simulink model "pd_plus_testings_7DOF_alternative"  (R2022b)
settings: Solver=ode4  StartTime=0.0  StopTime=101  FixedStep=1e-3  RelTol=1e-3
InitFcn:
  | parameters_7dof;
undefined symbols (not defined in the file): param_robot, q_0
(part 6 of 7)

== matlab function pd_plus_testings_7DOF_alternative/Subsystem/Coriolis Matrix ==
  data: q_state input; C output; q_state_dot input
function C = Franka_CoriolisMatrix(q_state, q_state_dot)
% Author: TU Wien, ACIN Robotics group
% Optimized and generated from Maple

  C = zeros(7,7);
  t2638 = q_state(7);
  t2624 = cos(t2638);
  t3209 = 0.10967182128164640000000000000000e-2 * t2624;
  t2617 = sin(t2638);
  t3260 = 0.33449653235675560000000000000000e-2 * t2617;
  t2102 = t3209 + t3260;
  t1973 = t2102 + 0.18713819462921000000000000000000e-3;
  t2639 = q_state(6);
  t2618 = sin(t2639);
  t3973 = t1973 * t2618;
  t1810 = t3973 - 0.30304889466540600000000000000000e-2;
  t3252 = 0.11357396418885000000000000000000e-1 * t2618;
  t2171 = -0.24178658687700000000000000000000e-2 + t3252;
  t2640 = q_state(5);
  t2619 = sin(t2640);
  t3206 = 0.12763550042100000000000000000000e-2 * t2624;
  t3271 = 0.51602752476000000000000000000000e-3 * t2617;
  t3723 = -t3271 - t3206;
  t3047 = -0.27219646194675000000000000000000e-1 + t3723;
  t2156 = 0.48418875570424600000000000000000e-2 * t2617 + 0.55042935974400000000000000000000e-3;
  t2610 = t2624 ^ 2;
  t2388 = 0.15804348732630080000000000000000e-2 * t2610;
  t2412 = 0.13614453378240000000000000000000e-2 * t2617;
  t3020 = 0.5826996021941340000000000000000e-3 - t2388 - t2412;
  t1748 = t2156 * t2624 + t3020;
  t4010 = t1748 * t2619;
  t1556 = t3047 - t4010;
  t2625 = cos(t2639);
  t4368 = t1556 * t2625;
  t1365 = t1810 * t2619 - t2171 + t4368;
  t2641 = q_state(4);
  t2627 = cos(t2641);
  t2613 = t2627 ^ 2;
  t4376 = t1365 * t2613;
  t2626 = cos(t2640);
  t4375 = t1365 * t2626;
  t2024 = t2102 + 0.187138194629210e-3;
  t1841 = t2024 * t2619 - 0.11357396418885000000000000000000e-1;
  t1801 = t1841 * t2625;
  t3249 = 0.52863517876992000000000000000000e-1 * t2618;
  t4130 = -0.33449653235675560000000000000000e-2 * t2624 + 0.10967182128164640000000000000000e-2 * t2617;
  t1838 = -t4130 + t3249 + 0.8968493211292842000000000000000e-2;
  t2107 = -0.66899306471351120000000000000000e-2 * t2624 + 0.21934364256329280000000000000000e-2 * t2617;
  t1967 = 0.22044137530701260000000000000000e-1 - t2107;
  t2611 = t2625 ^ 2;
  t3977 = t1967 * t2611;
  t3510 = t1838 - t3977;
  t2382 = 0.48152918111602840000000000000000e-2 * t2610;
  t3265 = 0.15804348732630080000000000000000e-2 * t2617;
  t2160 = -0.27228906756480000000000000000000e-2 + t3265;
  t2416 = 0.11008587194880000000000000000000e-2 * t2617;
  t2603 = t2617 ^ 2;
  t3573 = -t2160 * t2624 + t2416 + 0.26595745882176000000000000000000e-4 * t2603;
  t2986 = -0.11560955249855324000000000000000e-1 - t3573;
  t1663 = t2382 + t2986;
  t3194 = 0.59408523832320000000000000000000e-2 * t2624;
  t3262 = 0.24018735697920000000000000000000e-2 * t2617;
  t3718 = -t3262 - t3194;
  t3046 = -0.12669508046976000000000000000000e0 + t3718;
  t1513 = t1663 * t2618 + t3046;
  t4044 = t1513 * t2625;
  t1348 = t3510 - t4044;
  t4374 = t1348 * t2626;
  t4169 = -t4374 + t1801;
  t3201 = 0.24018735697920000000000000000000e-2 * t2624;
  t3729 = 0.59408523832320000000000000000000e-2 * t2617 - t3201;
  t4300 = 0.47796540830203740000000000000000e-1 - t3729;
  t4369 = t1556 * t2618;
  t2890 = t2619 * t4300 + t4169 - t4369 + 0.27752814537092170000000000000000e0;
  t4047 = t1348 * t2619;
  t3717 = -0.66899306471351120000000000000000e-2 * t2617 - 0.21934364256329280000000000000000e-2 * t2624;
  t2036 = t3717 * t2611;
  t2822 = t2036 + t2102;
  t3208 = 0.11008587194880000000000000000000e-2 * t2624;
  t3257 = 0.96837751140849200000000000000000e-2 * t2617;
  t2247 = t2624 * t3257;
  t3739 = -t2247 + t2388;
  t1704 = t2160 * t2617 + t3208 - t3739;
  t4326 = t1704 * t2618 - t3729;
  t4035 = t2625 * t4326;
  t4359 = t2822 - t4035;
  t1392 = t4359 * t2626;
  t2381 = 0.48418875570424600000000000000000e-2 * t2610;
  t3261 = 0.31608697465260160000000000000000e-2 * t2617;
  t2248 = t2624 * t3261;
  t2473 = 0.13614453378240000000000000000000e-2 * t2624;
  t3749 = t2248 - t2473;
  t1706 = -t2156 * t2617 + t2381 + t3749;
  t2413 = 0.12763550042100000000000000000000e-2 * t2617;
  t2480 = 0.51602752476000000000000000000000e-3 * t2624;
  t2111 = t2413 - t2480;
  t1564 = t1706 * t2619 - t2111;
  t4373 = -t1564 * t2618 - t1392;
  t2620 = sin(t2641);
  t1418 = t1513 * t2620 - t3047;
  t4046 = t1418 * t2625;
  t4372 = -t2171 - t4046;
  t2643 = q_state(2);
  t2629 = cos(t2643);
  t2642 = q_state(3);
  t2621 = sin(t2642);
  t2628 = cos(t2642);
  t2524 = 0.60149e-1 * t2625 + 0.14117e-1 * t2618;
  t3551 = 0.10517e-1 * t2626;
  t3300 = t2524 * t2619 + t3551;
  t2521 = 0.60149e-1 * t2618 - 0.14117e-1 * t2625;
  t2354 = t2521 + 0.384e0;
  t2226 = t2354 * t2620;
  t3558 = 0.10517e-1 * t2619;
  t2875 = -t2524 * t2626 + t3558;
  t2828 = 0.825e-1 + t2875;
  t4312 = t2627 * t2828;
  t3354 = -t2226 - t4312;
  t4331 = -0.825e-1 - t3354;
  t4341 = t2621 * t3300 + t2628 * t4331;
  t4250 = t2629 * t4341;
  t2622 = sin(t2643);
  t4237 = t4341 * t2622;
  t4001 = t1841 * t2618;
  t4370 = -t4001 - t4368;
  t4347 = t1748 * t2618;
  t1557 = t4300 + t4347;
  t1538 = t1557 * t2619;
  t2401 = 0.4815291811160284000000000000000e-2 * t2610;
  t2982 = 0.17806630741175110000000000000000e-1 + t3573;
  t1682 = t2982 - t2401;
  t3832 = t2618 * t2625;
  t4367 = (0.2e1 * t1682 - 0.12491350982639572000000000000000e-1) * t3832;
  t1664 = t2382 - t2982;
  t4366 = (0.2e1 * t1664 + 0.12491350982639572000000000000000e-1) * t3832;
  t3835 = t2618 * t2619;
  t4365 = (t1564 * t2625 + t3835 * t4130) * t2626;
  t2235 = 0.187138194629210e-3 + t3260;
  t3513 = t2625 * t3209 + t4347;
  t4364 = t2235 * t2625 + t3513;
  t2157 = 0.18713819462921000000000000000000e-3 + t3260;
  t4363 = t2157 * t2625 + t3513;
  t3694 = t1967 * t3832;
  t4025 = t1682 * t2611;
  t3319 = -t3694 - t4025;
  t2159 = 0.24209437785212300000000000000000e-2 * t2617 + 0.27521467987200000000000000000000e-3;
  t3898 = t2159 * t2617;
  t3204 = 0.15804348732630080000000000000000e-2 * t2624;
  t2249 = t2617 * t3204;
  t2385 = 0.24209437785212300000000000000000e-2 * t2610;
  t2477 = 0.68072266891200000000000000000000e-3 * t2624;
  t2854 = t2477 - t2385;
  t4210 = t2249 - t2854;
  t1707 = -t3898 + t4210;
  t4196 = t1707 * t2625;
  t4241 = t4130 * t2618;
  t1524 = t1706 * t2625 + t4241;
  t2612 = t2626 ^ 2;
  t4334 = t1524 * t2612;
  t4362 = t4334 - t4196;
  t3532 = 0.345563e0 * t2627;
  t3120 = 0.41065e-1 * t2619 + 0.11953e-1 * t2626;
  t2356 = t3120 + 0.825e-1;
  t3871 = t2356 * t2620;
  t3295 = -t3532 + t3871;
  t2046 = t3295 - 0.316e0;
  t2571 = 0.345563e0 * t2620;
  t3870 = t2356 * t2627;
  t4135 = t2571 + t3870;
  t4207 = -0.825e-1 + t4135;
  t2004 = t4207 * t2628;
  t3549 = 0.41065e-1 * t2626;
  t2522 = 0.11953e-1 * t2619 - t3549;
  t3820 = t2621 * t2522;
  t1785 = t2004 - t3820;
  t4002 = t1785 * t2622;
  t1578 = t2046 * t2629 - t4002;
  t2644 = q_state(1);
  t2630 = cos(t2644);
  t3160 = 0.61297300000000000000000000000000e0 * t2630;
  t3102 = t1578 * t3160;
  t4361 = 0.1e1 * t3102;
  t4358 = -t1524 * t2626 + t3723;
  t2604 = t2618 ^ 2;
  t2374 = 0.62456754913197860000000000000000e-2 * t2604;
  t3578 = t2249 + 0.16270818883971600000000000000000e-3 * t2603 - t2374;
  t1360 = t1664 * t2611 + t3578 + 0.50045957458821760000000000000000e-2 * t2610 - 0.12569364734109380000000000000000e-2 - t3694;
  t2033 = t2111 * t2618;
  t4342 = t1706 * t2618 + t3718;
  t4356 = -t2619 * t4342 + t2033;
  t2098 = 0.10517000000000000000000000000000e-1 * t2617 - 0.42520000000000000000000000000000e-2 * t2624;
  t2037 = t2098 * t2619;
  t2128 = 0.10517000000000000000000000000000e-1 * t2624 + 0.42520000000000000000000000000000e-2 * t2617;
  t1966 = 0.88000000000000000000000000000000e-1 + t2128;
  t3248 = 0.61597000000000000000000000000000e-1 * t2618;
  t3793 = t2625 * t2626;
  t3760 = t1966 * t3793 + t2626 * t3248;
  t4156 = t2037 + t3760;
  t1561 = 0.82500000000000000000000000000000e-1 - t4156;
  t4353 = t1561 * t2620;
  t4352 = t1561 * t2627;
  t3972 = t1973 * t2625;
  t4350 = t3972 + t4347;
  t4346 = t1748 * t2625;
  t1506 = t4346 - t1810;
  t2523 = 0.39252e-1 * t2628 + 0.27518e-1 * t2621;
  t2623 = sin(t2644);
  t3117 = 0.39252e-1 * t2621 - 0.27518e-1 * t2628;
  t2871 = t3117 * t2629 - 0.249498e0 * t2622;
  t4324 = t2523 * t2623 + t2630 * t2871;
  t4349 = 0.1e1 * t4324;
  t4322 = 0.1e1 * t2623;
  t3897 = t2159 * t2624;
  t2390 = 0.79021743663150400000000000000000e-3 * t2610;
  t2419 = 0.68072266891200000000000000000000e-3 * t2617;
  t2883 = -0.29134980109706700000000000000000e-3 + t2419;
  t4133 = t2883 + t2390;
  t1744 = t3897 - t4133;
  t2423 = 0.25801376238000000000000000000000e-3 * t2617;
  t2478 = 0.63817750210500000000000000000000e-3 * t2624;
  t3724 = t2423 + t2478;
  t1962 = -t3724 - 0.13609823097337500000000000000000e-1;
  t3985 = t1962 * t2619;
  t1549 = t1744 - t3985;
  t4348 = t1549 * t2625;
  t1643 = t1663 * t2611;
  t3958 = t3047 * t2625;
  t1755 = t3958 - t2171;
  t4345 = t1755 * t2619;
  t1726 = t1755 * t2626;
  t4344 = t1785 * t2629;
  t3791 = t2626 * t2620;
  t2420 = 0.63817750210500000000000000000000e-3 * t2617;
  t3216 = 0.25801376238000000000000000000000e-3 * t2624;
  t2119 = t3216 - t2420;
  t3044 = -0.55993270925625000000000000000000e-2 - t2119;
  t4343 = t3044 * t2626;
  t1552 = -t2619 * t3047 + t1748;
  t1672 = t1704 * t2611;
  t2001 = t3717 * t3832;
  t3317 = -t2001 - t1672;
  t3789 = t2626 * t2628;
  t4340 = 0.1e1 * t3789;
  t4339 = 0.1e1 * t4345;
  t3263 = 0.23920000000000000000000000000000e-2 * t2617;
  t2338 = 0.682e-3 + t3263;
  t3205 = 0.14820000000000000000000000000000e-2 * t2624;
  t2387 = 0.17120000000000000000000000000000e-2 * t2610;
  t3838 = t2617 * t2624;
  t3087 = 0.49780000000000000000000000000000e-2 * t3838;
  t2826 = t3087 - t2387;
  t1885 = t2826 - 0.14600000000000000000000000000000e-2;
  t3990 = t1885 * t2625;
  t3764 = -t2618 * t3205 + t3990;
  t3585 = -t2338 * t2618 + t3764;
  t1618 = 0.4234e-2 + t3585;
  t3826 = t2619 * t2626;
  t1581 = t1618 * t3826;
  t3565 = 0.5317e-1 * t2620;
  t2563 = -0.316e0 + t3565;
  t3533 = 0.104419e0 * t2627;
  t3119 = 0.104419e0 * t2620 + 0.5317e-1 * t2627;
  t2357 = t3119 - 0.825e-1;
  t2088 = t2357 * t2628 - 0.27454e-1 * t2621;
  t4259 = t2088 * t2629;
  t1767 = t4259 + t2622 * (t2563 - t3533);
  t4338 = t1767 * t2630;
  t2414 = 0.12009367848960000000000000000000e-2 * t2617;
  t2161 = t2414 + 0.63347540234880000000000000000000e-1;
  t2469 = 0.29704261916160000000000000000000e-2 * t2624;
  t1978 = -t2469 - t2161;
  t4337 = t1978 * t2625;
  t3091 = 0.17120000000000000000000000000000e-2 * t3838;
  t3273 = 0.49780000000000000000000000000000e-2 * t2610;
  t2825 = t3091 + t3273;
  t1897 = 0.5644000000000000000000000000000e-2 + t2825;
  t1854 = t1897 * t2611;
  t2848 = -0.47840000000000000000000000000000e-2 * t2624 + 0.29640000000000000000000000000000e-2 * t2617;
  t2065 = -0.436e-3 + t2848;
  t1948 = t2065 * t3832;
  t3762 = t1854 + t1948;
  t1486 = t2825 + t3762 - 0.5410000000000000000000000000000e-2;
  t2605 = t2619 ^ 2;
  t3711 = -0.1e1 * t2605 + t2612;
  t4336 = t3711 * t1486;
  t2422 = 0.54835910640823200000000000000000e-3 * t2617;
  t3203 = 0.16724826617837780000000000000000e-2 * t2624;
  t2852 = -t3203 + t2422;
  t4248 = t2852 * t2618;
  t4335 = t4248 * t2627;
  t3289 = 0.4841887557042460000000000000000e-2 * t2617;
  t2200 = 0.55042935974400000000000000000000e-3 + t3289;
  t1749 = -t2200 * t2624 - t3020;
  t1559 = -t1749 * t2618 + t4300;
  t4333 = t1559 + t3972;
  t4319 = t1707 * t2619;
  t4332 = t2119 + t4319;
  t3269 = 0.79021743663150400000000000000000e-3 * t2617;
  t2250 = t2624 * t3269;
  t3748 = t2250 + 0.25022978729410880000000000000000e-2 * t2610;
  t3121 = 0.6284682367054690000000000000000e-3 - t3748;
  t4330 = 0.81354094419858000000000000000000e-4 * t2603 - t3121;
  t2002 = 0.3742763892584200000000000000000e-3 - t3717;
  t3953 = t2002 * t2625;
  t2155 = 0.11008587194880000000000000000000e-2 + t3257;
  t2383 = 0.31608697465260160000000000000000e-2 * t2610;
  t2408 = 0.27228906756480000000000000000000e-2 * t2617;
  t4282 = t2383 + t2408 - 0.11653992043882680000000000000000e-2;
  t1742 = -t2155 * t2624 + t4282;
  t4318 = t1742 * t2618;
  t4329 = t3953 - t4318;
  t3932 = t2620 * t2828;
  t4328 = t3932 - 0.316e0;
  t3552 = 0.61597e-1 * t2625;
  t2527 = 0.10517e-1 * t2624 + 0.4252e-2 * t2617;
  t2359 = t2527 + 0.88e-1;
  t3869 = t2359 * t2618;
  t2834 = -t3552 + t3869;
  t4105 = 0.384e0 + t2834;
  t4242 = t4105 * t2627;
  t4274 = -t4242 - 0.316e0;
  t4243 = t4105 * t2620;
  t4106 = 0.825e-1 - t4243;
  t4327 = t1486 * t3826 + t3585 + 0.6898e-2;
  t1968 = 0.11022068765350630000000000000000e-1 - t4130;
  t2421 = 0.55042935974400000000000000000000e-3 * t2617;
  t3725 = t2421 + t2473;
  t1971 = 0.89166132435286430000000000000000e-2 + t3725;
  t3790 = t2626 * t2627;
  t1603 = t1968 * t3790 - t1971 * t2620;
  t2168 = 0.76800000000000000000000000000000e0 * t2618 + 0.17600000000000000000000000000000e0;
  t2410 = 0.24444132201840000000000000000000e-2 * t2617;
  t3211 = 0.98827089590400000000000000000000e-3 * t2624;
  t4222 = -t3211 + t2410;
  t2812 = t2618 * t4222;
  t3451 = 0.7735484874e-2 * t2617;
  t3834 = t2618 * t2620;
  t4323 = t2119 * t3834 + t2168 * t3451 + t2627 * t2812;
  t2306 = t2625 * t3205;
  t3991 = t1885 * t2618;
  t1623 = t2338 * t2625 + t2306 + t3991;
  t4321 = t1623 * t3826;
  t4320 = t1707 * t2618;
  t4317 = t1744 * t2618;
  t1720 = t1744 * t2619;
  t4316 = t1744 * t2620;
  t4315 = t1744 * t2621;
  t4016 = t1744 * t2625;
  t4014 = t1744 * t2626;
  t3786 = t2627 * t2625;
  t4314 = t1744 * t3786;
  t3787 = t2627 * t2618;
  t4313 = t1744 * t3787;
  t3548 = 0.61597e-1 * t2626;
  t2537 = t2618 * t3548;
  t3123 = 0.10517e-1 * t2617 - 0.4252e-2 * t2624;
  t4256 = t2619 * t3123;
  t4122 = -t2359 * t3793 - t4256;
  t1775 = t2537 - 0.825e-1 - t4122;
  t4005 = t1775 * t2620;
  t4004 = t1775 * t2627;
  t2509 = 0.11357396418885000000000000000000e-1 * t2625;
  t3961 = t3047 * t2618;
  t4217 = -t3961 - t2509;
  t1771 = t2626 * t4217;
  t3559 = 0.61597e-1 * t2618;
  t3301 = t2359 * t2625 + t3559;
  t4245 = t3123 * t2626;
  t2741 = t2619 * t3301 - t4245;
  t4311 = t2741 * t2621;
  t4310 = t2741 * t2628;
  t3669 = t1897 * t3832;
  t3934 = t2065 * t2611;
  t4108 = t2065 * t2604 + 0.2e1 * t3669 - t3934;
  t4309 = -t3826 * t4108 - t1623;
  t1939 = t2159 * t2618 + 0.12009367848960000000000000000000e-2;
  t2407 = 0.29704261916160000000000000000000e-2 * t2617;
  t2158 = t2407 - 0.23898270415101870000000000000000e-1;
  t2268 = t2618 * t2390;
  t1531 = t1939 * t2624 - t2618 * t2883 - t2158 - t2268;
  t2609 = t2623 ^ 2;
  t2616 = t2630 ^ 2;
  t4134 = t2616 + t2609;
  t1935 = t2002 * t2618;
  t3155 = -t1742 * t2625 + 0.60609778933081200000000000000000e-2;
  t1507 = t3155 - t1935;
  t3290 = 0.4841887557042460000000000000000e-2 * t2610;
  t4307 = -t3290 - t3749;
  t2375 = 0.31228377456598930000000000000000e-2 * t2604;
  t3747 = t2250 + t2385;
  t4306 = t3747 - t2375;
  t3053 = 0.33106000000000000000000000000000e-1 - t2825;
  t2471 = 0.23920000000000000000000000000000e-2 * t2624;
  t3266 = 0.14820000000000000000000000000000e-2 * t2617;
  t3720 = -t3266 + t2471;
  t2063 = -0.218e-3 - t3720;
  t3666 = t2063 * t3832;
  t3092 = 0.85600000000000000000000000000000e-3 * t3838;
  t3274 = 0.24890000000000000000000000000000e-2 * t2610;
  t2018 = t3092 + t3274;
  t1884 = t2018 + 0.28220000000000000000000000000000e-2;
  t3992 = t1884 * t2611;
  t3763 = -t3992 - t3666;
  t4305 = t3763 - t3053;
  t3909 = t2119 * t2627;
  t4304 = -t3909 + t2119;
  t3291 = 0.2420943778521230000000000000000e-2 * t2610;
  t3449 = 0.7735484874e-2 * t2624;
  t3347 = t2168 * t3449;
  t4302 = (t3291 + 0.790217436631504e-3 * t3838 - 0.6002993810686607000000000000000e-2) * t2612 - 0.1e1 * t3347;
  t2573 = 0.249498e0 * t2629;
  t4183 = t2622 * t3117;
  t4281 = t2573 + t4183;
  t4301 = 0.3228604e1 * t4281;
  t3214 = 0.54835910640823200000000000000000e-3 * t2624;
  t3264 = 0.16724826617837780000000000000000e-2 * t2617;
  t3719 = -t3264 - t3214;
  t2025 = -t3719 + 0.93569097314605e-4;
  t4299 = 0.1e1 * t1744;
  t4298 = t2627 - 0.1e1;
  t1813 = -t1973 * t2619 + 0.11357396418885000000000000000000e-1;
  t4296 = t1813 * t2618;
  t3275 = 0.85600000000000000000000000000000e-3 * t2610;
  t1857 = 0.85600000000000000000000000000000e-3 * t2603 + t3087 - t3275;
  t2106 = t3205 + t3263;
  t3664 = t2106 * t3832;
  t3999 = t1857 * t2611;
  t3765 = t3999 - t3664;
  t4160 = t1857 + t3765;
  t4295 = t2612 * t4160;
  t3817 = t2621 * t2620;
  t3813 = t2621 * t2627;
  t4294 = t2621 * t4207;
  t2845 = t2622 * t2875;
  t3783 = t2628 * t2627;
  t2204 = t2522 * t3783;
  t4104 = t2621 * t3120 + t2204;
  t4293 = t2622 * t4104;
  t3798 = t2625 * t2619;
  t3329 = -t2359 * t3798 - t2619 * t3559 + t4245;
  t4290 = t3329 * t2621;
  t4003 = t3329 * t2628;
  t4288 = (t2621 * t3123 + t3301 * t3783) * t2619;
  t2386 = 0.24076459055801420000000000000000e-2 * t2610;
  t3731 = -t2386 + t2421;
  t2162 = -0.13614453378240000000000000000000e-2 + t3269;
  t3892 = t2162 * t2624;
  t2980 = 0.89033153705875550000000000000000e-2 - t3892 + t3731;
  t3402 = 0.13297872941088e-4 * t2603;
  t1696 = t2980 + t3402;
  t4287 = t1696 * t2611 + 0.3122837745659893e-2 * t2604;
  t3945 = t2046 * t2622;
  t1572 = t3945 + t4344;
  t3195 = 0.48418875570424600000000000000000e-2 * t2624;
  t2827 = t2617 * t3195 - t2390;
  t3279 = 0.79021743663150400000000000000000e-3 * t2603;
  t1858 = t2827 + t3279;
  t2479 = 0.55042935974400000000000000000000e-3 * t2624;
  t3893 = t2162 * t2617;
  t1710 = -t2827 - t2479 - t3893;
  t1678 = t1710 * t2611;
  t3665 = t2102 * t3832;
  t4124 = t3665 + t1678;
  t4286 = -t1858 + t4124;
  t2027 = t2102 * t2611;
  t1677 = t1710 * t2618;
  t2474 = 0.12009367848960000000000000000000e-2 * t2624;
  t2103 = t2407 - t2474;
  t4164 = t1677 + t2103;
  t4036 = t4164 * t2625;
  t4285 = -t2027 + t4036;
  t2112 = t2414 + t2469;
  t4247 = t2852 * t2625;
  t4284 = -t2112 - t4247;
  t1940 = t2162 * t2618 - 0.29704261916160000000000000000000e-2;
  t4283 = -t1940 * t2624 + t2161;
  t1807 = 0.175156065026714e-3 - t4306;
  t3709 = -0.2e1 * t3826;
  t2179 = 0.11198654185125000000000000000000e-1 - t2413;
  t1989 = t2480 + t2179;
  t3956 = t1989 * t2626;
  t3758 = 0.46660838454822060000000000000000e-2 * t3826 + t3956;
  t4279 = t3758 + t1807 * t3709 - 0.1e1 * t4345;
  t3873 = t2354 * t2627;
  t4278 = t3873 - t3932;
  t3369 = -t3565 + t3533;
  t2355 = -t3369 - 0.316e0;
  t1791 = -t2355 * t2622 - t4259;
  t4276 = -0.1e1 * t2603 + t2610;
  t4275 = -0.1e1 * t3897 + t4133;
  t3130 = 0.2872e-1 * t2622 - 0.3141e-2 * t2629;
  t4272 = 0.646926e0 * t3130;
  t3153 = -t3961 + 0.27752814537092170000000000000000e0;
  t4271 = t1813 * t2625 - t3153;
  t2184 = -0.65933151443131591200000000000000e0 - t2421;
  t3268 = 0.98827089590400000000000000000000e-3 * t2617;
  t2182 = -0.52129746651620000000000000000000e-1 - t3268;
  t3199 = 0.24444132201840000000000000000000e-2 * t2624;
  t3022 = t2182 - t3199;
  t2810 = t2618 * t3022 - 0.50330438027992300000000000000000e0;
  t4089 = 0.13609823097337500000000000000000e-1 + t2423;
  t4138 = t2478 + t4089;
  t2811 = t4138 * t2618 + 0.29682175996164750000000000000000e0;
  t4269 = t2620 * t2811 + t2627 * t2810 + t2184;
  t3184 = 0.52863517876992000000000000000000e-1 * t2625;
  t4268 = t2018 - 0.27050000000000000000000000000000e-2;
  t1970 = -t2852 + 0.44842466056464210000000000000000e-2;
  t3238 = 0.12089329343850000000000000000000e-2 * t2620;
  t3715 = -t1970 * t2627 - t3238;
  t2823 = -0.46305794820080000000000000000000e-2 - t3715;
  t3050 = -0.21447119530300000000000000000000e-1 + t4222;
  t2114 = t3199 + t3268;
  t1986 = t2114 + 0.52129746651620000000000000000000e-1;
  t3971 = t3044 * t2619;
  t1605 = t1986 * t2618 - t3971 + 0.58416762559717300000000000000000e0;
  t4266 = t1605 * t2627;
  t3975 = t1968 * t2618;
  t1809 = 0.52863517876992000000000000000000e-1 + t3975;
  t4265 = t1809 * t2625;
  t4264 = t1940 * t2617;
  t4260 = t2088 * t2622;
  t4258 = t2161 * t2618;
  t4257 = t2612 * t3783;
  t4255 = t2621 * t3301;
  t4253 = t2623 * t3130;
  t4232 = -t2386 - t3892;
  t3581 = -t2421 - t4232;
  t2984 = -0.57804776249276620000000000000000e-2 + t3581;
  t1694 = -t3402 + t2984;
  t1660 = t1694 * t2618;
  t4166 = t1660 + t1978;
  t4252 = t2626 * t4166;
  t4251 = t2629 * t4135;
  t3818 = t2621 * t2619;
  t4249 = t2834 * t3818;
  t4173 = t3123 * t3834;
  t3782 = t2629 * t2620;
  t4244 = t3300 * t3782;
  t2005 = t3300 * t3783;
  t3810 = t2622 * t2620;
  t4172 = t3300 * t3810;
  t1998 = t4130 * t3798;
  t3255 = 0.14600000000000000000000000000000e-2 * t2618;
  t2062 = t2106 + 0.682e-3;
  t3938 = t2062 * t2625;
  t4148 = t2618 * t2826 - t3255 + t3938 - 0.458e-3;
  t4240 = t4148 * t2619;
  t4239 = t4148 * t2626;
  t4238 = t4331 * t2621;
  t2075 = t2171 * t2619;
  t1657 = t2075 - t3973 - 0.47802211058981400000000000000000e-2;
  t4236 = -t1507 * t2612 + t1657;
  t2367 = 0.13297872941088000000000000000000e-4 * t2603;
  t2983 = -0.89033153705875550000000000000000e-2 + t3581;
  t1666 = -t2367 + t2983;
  t1639 = t1666 * t2611;
  t1728 = -t2375 + t4330;
  t4235 = t1728 + t1639;
  t3090 = 0.24890000000000000000000000000000e-2 * t3838;
  t1882 = t3090 - 0.73000000000000000000000000000000e-3 - t3275;
  t3997 = t1882 * t2618;
  t1827 = 0.229e-3 - t3997;
  t3213 = 0.74100000000000000000000000000000e-3 * t2624;
  t3267 = 0.11960000000000000000000000000000e-2 * t2617;
  t2851 = -t3213 - t3267;
  t2064 = t2851 - 0.341e-3;
  t3935 = t2064 * t2625;
  t1609 = t1827 + t3935;
  t3018 = t2479 - t2390;
  t1705 = (t2162 + t3195) * t2617 + t3018;
  t1525 = t1705 * t2611 - t3665;
  t1414 = t1858 + t1525;
  t3231 = 0.82500000000000000000000000000000e-1 * t2620;
  t2175 = 0.38400000000000000000000000000000e0 - t3231;
  t2019 = t2175 * t3449;
  t3452 = 0.3127439544e-2 * t2617;
  t3346 = t2175 * t3452;
  t4234 = -t2019 - 0.63347540234880000000000000000000e-1 - t3346;
  t2246 = 0.99560000000000000000000000000000e-2 * t3838;
  t1855 = t2246 - t2387 + 0.17120000000000000000000000000000e-2 * t2603;
  t3957 = t1989 * t2619;
  t4152 = t2249 + t3957;
  t2378 = 0.23330419227411030000000000000000e-2 * t2605;
  t4233 = -t2378 - t2381;
  t4231 = -t2479 + t2412;
  t4229 = t1973 * t3798 - t2509;
  t2513 = 0.12089329343850000000000000000000e-2 * t2627;
  t4228 = -t2513 - 0.46305794820080000000000000000000e-2 * t2620;
  t2173 = -0.31600000000000000000000000000000e0 * t2620 + 0.82500000000000000000000000000000e-1;
  t2512 = 0.21751134959804000000000000000000e-1 * t2626;
  t2768 = t1962 + t2512;
  t2757 = t2768 * t2627;
  t2967 = t3449 + t3452;
  t4227 = t2967 * t2173 + t1720 + t2757 + 0.13609823097337500000000000000000e-1;
  t3151 = t2422 - 0.44842466056464210000000000000000e-2;
  t2769 = 0.46305794820080000000000000000000e-2 * t2627 + t3151 - t3238;
  t4226 = t2769 - t3203;
  t2599 = 0.316e0 * t2622;
  t1400 = t2622 * t4278 + t2599 - t4250;
  t2841 = t3300 * t2628;
  t1575 = -t2841 + t4238;
  t4034 = t1575 * t2623;
  t1287 = t1400 * t2630 + t4034;
  t3131 = -0.1e1 * t3873 + t4328;
  t1401 = t2622 * t3131 + t4250;
  t4033 = t1575 * t2630;
  t1289 = t1401 * t2623 + t4033;
  t3158 = 0.83327750000000000000000000000000e0 * t2630;
  t3218 = 0.83327750000000000000000000000000e0 * t2623;
  t4225 = t1287 * t3218 + t1289 * t3158;
  t3183 = 0.61597000000000000000000000000000e-1 * t2625;
  t3979 = t1966 * t2618;
  t2951 = -t3183 + t3979;
  t1753 = t2951 + 0.38400000000000000000000000000000e0;
  t1725 = t1753 * t2620;
  t1714 = -0.825e-1 + t1725;
  t1589 = 0.825e-1 - t4156;
  t4029 = t1589 * t2627;
  t3040 = -t4290 + (t1714 + t4029) * t2628;
  t1315 = t3040 * t2623;
  t3571 = 0.825e-1 * t2621;
  t2556 = t2630 * t3571;
  t3359 = t1725 + t4029;
  t4030 = t1589 * t2620;
  t3521 = t4030 + t4274;
  t3376 = t3521 * t2622;
  t1152 = t1315 * t2629 - t2556 + t2623 * t3376 + (t2621 * t3359 + t4003) * t2630;
  t3408 = -t1966 * t3798 - t2619 * t3248;
  t1648 = t4245 + t3408;
  t3410 = t1648 * t2621 + t1775 * t3783 + t2628 * t4106;
  t1351 = t3410 * t2630;
  t3357 = t4243 - t4004;
  t3515 = t4005 - t4274;
  t3375 = t3515 * t2630;
  t4028 = t1648 * t2628;
  t1187 = t1351 * t2629 + t2622 * t3375 + (t4028 + (t3357 - 0.825e-1) * t2621) * t2623;
  t3161 = 0.36776100000000000000000000000000e0 * t2630;
  t3221 = 0.36776100000000000000000000000000e0 * t2623;
  t4224 = t1152 * t3161 + t1187 * t3221;
  t3292 = 0.7902174366315040000000000000000e-3 * t2610;
  t4221 = t3292 + t2883;
  t2038 = t2098 * t2626;
  t4220 = t3408 + t2038;
  t2740 = t2626 * t3301 + t4256;
  t2734 = 0.825e-1 - t2740;
  t2706 = t2620 * t2734 + t4274;
  t3542 = 0.735522e0 * t2706 * t2629 + 0.735522e0 * (-t4311 + ((-0.825e-1 + t2740) * t2627 + t4106) * t2628) * t2622;
  t4125 = t4134 * t3542;
  t2464 = 0.54835910640823200000000000000000e-3 * t2621;
  t3422 = 0.2444413220184e-2 * t2628;
  t3713 = -t3422 + t2464;
  t3434 = 0.6381775021050e-3 * t2620;
  t2949 = 0.2444413220184e-2 * t2627 - t3434;
  t4219 = t2604 * t4231 - t3665;
  t3544 = 0.27454e-1 * t2628;
  t2087 = t2357 * t2621 + t3544;
  t3930 = t2087 * t2623;
  t1576 = t3930 - t4338;
  t3116 = t2087 * t2630;
  t1582 = t1767 * t2623 + t3116;
  t4216 = t1576 * t2623 + t1582 * t2630;
  t3401 = 0.81354094419858e-4 * t2603;
  t3667 = t1968 * t3832;
  t4215 = -t3401 + t3667 + t4287;
  t4213 = t2387 - 0.1e1 * t3087;
  t2725 = -t3873 + t4328;
  t1274 = t2629 * t2725 - t4237;
  t3497 = 0.1666555e1 * t1274;
  t3399 = t2616 * t3497;
  t3400 = t2609 * t3497;
  t4113 = -0.1e1 * t3399 - 0.1e1 * t3400;
  t4211 = -0.1e1 * t1287 * t2623 - 0.1e1 * t1289 * t2630;
  t3089 = 0.48152918111602840000000000000000e-2 * t3838;
  t4209 = -t2618 * t3089 + t2268 - t2474;
  t4200 = t2367 + 0.32797153116247448000000000000000e-1;
  t3043 = -t2421 - t4200;
  t3800 = t2624 * t2626;
  t4208 = t2162 * t3800 + (t2386 + t3043) * t2626;
  t2569 = 0.3507900e-3 * t2619;
  t3283 = 0.925496e-3 + t2569;
  t4206 = 0.735522e0 * t3283;
  t4205 = -t1939 * t2617 - t2469;
  t2201 = 0.9356909731460500000000000000000e-4 + t3264;
  t3241 = 0.50000000000000000000000000000000e0 * t2619;
  t4198 = t2626 * t4089 - 0.21751134959804000000000000000000e-1;
  t4197 = -0.36776100000000000000000000000000e0 * t1152 * t2630 - 0.36776100000000000000000000000000e0 * t1187 * t2623;
  t4083 = 0.2e1 * t2618;
  t1859 = -0.49780000000000000000000000000000e-2 * t2603 + t3273 + 0.34240000000000000000000000000000e-2 * t3838;
  t4195 = t1859 * t2618;
  t1860 = -0.24890000000000000000000000000000e-2 * t2603 + t3091 + t3274;
  t4194 = t1860 * t2618;
  t4193 = t2158 * t2628;
  t2165 = 0.55993270925625000000000000000000e-2 - t2420;
  t4192 = t2165 * t2627;
  t2928 = t2359 * t2620;
  t3572 = 0.825e-1 * t2620;
  t3321 = -0.316e0 + t3572;
  t2361 = 0.384e0 * t2627 - t3321;
  t4191 = t2361 * t2625;
  t4190 = t2523 * t2622;
  t4058 = t2629 / 0.2e1;
  t3628 = t2611 * t4058;
  t4189 = t2612 * t2620;
  t3784 = t2628 * t2620;
  t3596 = t3784 / 0.2e1;
  t3465 = t2612 * t3596;
  t3563 = 0.4252e-2 * t2626;
  t4188 = t2617 * (t2625 * t3558 + t3563);
  t4187 = t2618 * t2848;
  t3439 = 0.11953e-1 * t3783;
  t4186 = t2619 * (0.41065e-1 * t2621 + t3439);
  t3823 = t2620 * t2619;
  t4182 = t2622 * t3119;
  t3566 = 0.4252e-2 * t2619;
  t4181 = t2624 * (t2625 * t3566 - t3551);
  t3797 = t2625 * t2620;
  t4180 = t2625 * (0.68480000000000000000000000000000e-2 * t3838 + 0.99560000000000000000000000000000e-2 * t4276);
  t2999 = 0.41065e-1 * t3783 - 0.11953e-1 * t2621;
  t4179 = t2626 * t2999;
  t2776 = t2617 * (t2625 * t3551 - t3566) - t2624 * (t2625 * t3563 + t3558);
  t4178 = t2627 * t2776;
  t2709 = t2627 * t2734 + t4243;
  t1160 = t2706 * t2622 + (t4311 + (-0.825e-1 + t2709) * t2628) * t2629;
  t3529 = 0.345563e0 * t2629;
  t2533 = t2627 * t3529;
  t3570 = 0.825e-1 * t2627;
  t2565 = 0.825e-1 - t3570;
  t3537 = 0.345563e0 * t2622;
  t3413 = t2628 * t3537;
  t3806 = t2622 * t2628;
  t3808 = t2622 * t2626;
  t3809 = t2622 * t2621;
  t3828 = t2619 * t2622;
  t1397 = -t2565 * t3806 + t2620 * t3413 - t2629 * t3321 + t2999 * t3828 - t3120 * t3782 + t3439 * t3808 + t3549 * t3809 + t2533;
  t3530 = 0.104419e0 * t2629;
  t4121 = t2563 * t2629 - t2627 * t3530;
  t1646 = -t4260 + t4121;
  t2528 = 0.2872e-1 * t2629 + 0.3141e-2 * t2622;
  t2636 = q_state_dot(2);
  t3491 = 0.3228604e1 * t2871;
  t3492 = 0.3587895e1 * t1791;
  t3494 = 0.1225946e1 * t3945 + 0.1225946e1 * (t2004 - 0.1e1 * t3820) * t2629;
  t3496 = 0.1666555e1 * t2725 * t2622 + 0.1666555e1 * t4250;
  t4177 = (t1160 * t3542 + t1274 * t3496 - t1397 * t3494 - t1646 * t3492 + t2528 * t4272 - t3491 * t4281) * t2636;
  t3311 = t2521 * t3791 - t2524 * t2627;
  t4171 = t3311 * t2622;
  t3312 = t2521 * t3790 + t2524 * t2620;
  t1852 = t3312 * t2628;
  t4170 = t3909 * t2625;
  t3152 = t2421 + 0.57804776249276620000000000000000e-2;
  t1956 = t2367 + t3152;
  t2987 = -t2386 * t2618 + t4283;
  t1484 = t1956 * t2618 + t2987;
  t1903 = t1962 * t2620;
  t1388 = t1484 * t2627 + t1903;
  t3948 = t2024 * t2625;
  t4168 = t1557 + t3948;
  t1668 = t2367 + t2980;
  t4167 = t1668 * t2611 + t2375;
  t2274 = t2618 * t3209;
  t4163 = t4346 - t2274;
  t1824 = t1859 * t2625;
  t4161 = -t2618 * t3266 - t1824;
  t1914 = t3044 * t2627;
  t3982 = t3050 * t2620;
  t4159 = -t1914 - t3982;
  t4158 = -t1986 - t1903;
  t3234 = 0.13609823097337500000000000000000e-1 * t2620;
  t4157 = t3234 + t4234;
  t4150 = -t2250 - t3291;
  t2304 = t2619 * t2509;
  t4149 = t2304 - t3972;
  t2363 = 0.15804348732630080000000000000000e-2 * t2603;
  t3916 = t3723 * t2619;
  t4145 = -t2363 + t3916;
  t3727 = 0.25527100084200000000000000000000e-2 * t2617 - 0.10320550495200000000000000000000e-2 * t2624;
  t2451 = 0.26431758938496000000000000000000e-1 * t2618;
  t3851 = t2611 * t1968;
  t4140 = t2451 - t3851;
  t2518 = 0.16724826617837780000000000000000e-2 * t2628;
  t2205 = -t2518 - 0.988270895904e-3 * t2621;
  t3166 = 0.49096519673609460000000000000000e-2 * t2628;
  t3057 = t2627 * t3166;
  t3243 = 0.49096519673609460000000000000000e-2 * t2619;
  t4131 = t2621 * t3243 - t2626 * t3057;
  t1902 = t1962 * t2618;
  t3983 = t3050 * t2619;
  t1604 = -0.12908973617152500000000000000000e-1 + t3983 - t1902;
  t3207 = 0.11960000000000000000000000000000e-2 * t2624;
  t3270 = 0.74100000000000000000000000000000e-3 * t2617;
  t2115 = -t3207 + t3270;
  t4126 = 0.3587895e1 * t4134 * t1646;
  t2320 = t2527 * t2626;
  t4123 = -t3123 * t3798 - t2320;
  t3858 = t2604 * t1968;
  t3508 = t3851 - t3858;
  t1965 = -t2162 + 0.29704261916160000000000000000000e-2 * t2618;
  t4119 = t1965 * t2624 + t4258;
  t3937 = t2063 * t2611;
  t3503 = t2063 * t2604 - t3937;
  t2606 = t2620 ^ 2;
  t4118 = t2613 - 0.1e1 * t2606;
  t4117 = -0.1e1 * t4238 + t2841;
  t2122 = -0.41065000000000000000000000000000e-1 * t2626 + 0.11953000000000000000000000000000e-1 * t2619;
  t3906 = t2122 * t2621;
  t4116 = -0.1e1 * t3906 + t2004;
  t4115 = -0.1e1 * t1639 - 0.1e1 * t1728;
  t3495 = 0.1225946e1 * t1397;
  t3395 = t2616 * t3495;
  t3396 = t2609 * t3495;
  t4114 = -0.1e1 * t3396 - 0.1e1 * t3395;
  t1406 = t4286 * t2612;
  t1821 = t1858 * t2611;
  t3732 = t2363 - t2388;
  t1856 = t2247 + t3732;
  t4112 = t1406 - t1821 + t1856 - t3916 - t4219 + t4365;
  t4111 = t3121 + t4215;
  t2762 = t3992 + t4268;
  t1480 = t3666 + t2762;
  t1599 = t1618 * t2612;
  t3788 = t2626 * t2629;
  t3656 = t2619 * t3788;
  t3780 = t2629 * t2625;
  t4110 = t1480 * t3656 - t1599 * t2629 + t1882 * t3780;
  t3302 = t2235 * t2618 - 0.3030488946654060e-2;
  t1519 = -t3302 + t4163;
  t3384 = 0.1644487577369270e-2 * t2620;
  t3845 = t2612 * t2627;
  t4109 = t1519 * t3845 + t3384 - t4314;
  t3378 = -t2627 * t4206 + 0.735522e0 * t2569;
  t3481 = 0.8676525e-3 * t2619;
  t2557 = -0.374176e-3 + t3481;
  t2351 = t2557 * t2627;
  t3379 = 0.735522e0 * t2351 - 0.735522e0 * t3481;
  t3190 = 0.16724826617837780000000000000000e-2 * t2625;
  t3705 = 0.88e-1 * t2618;
  t2568 = 0.384e0 + t3705;
  t3453 = 0.7735484874e-2 * t2568;
  t2901 = -t3190 + t3453;
  t3427 = 0.6381775021050e-3 * t2627;
  t4103 = -t2620 * t2901 - t3427;
  t4102 = t2621 * t3119 + t3544;
  t4101 = 0.988270895904e-3 * t2620;
  t3426 = 0.1200936784896e-2 * t2627;
  t3016 = 0.988270895904e-3 + t3426;
  t4099 = t4346 + 0.3030488946654060e-2;
  t3949 = t2024 * t2618;
  t3304 = -0.3030488946654060e-2 + t3949;
  t1529 = -t4346 + t3304;
  t4039 = t1529 * t2612;
  t4098 = t4039 - 0.2390110552949070e-2;
  t3230 = 0.63817750210500000000000000000000e-3 * t2621;
  t1861 = -t2159 * t3789 - t3230;
  t4097 = t1861 * t2624 + t3789 * t4221;
  t3546 = 0.60149e-1 * t2627;
  t3547 = 0.14117e-1 * t2627;
  t3555 = 0.60149e-1 * t2620;
  t3556 = 0.14117e-1 * t2620;
  t4096 = t2618 * (t2626 * t3555 - t3547) - t2625 * (t2626 * t3556 + t3546);
  t4094 = 0.50000000000000000000000000000000e0 * t2612;
  t4093 = 0.83327750000000000000000000000000e0 * t2622;
  t4092 = 0.17939475000000000000000000000000e1 * t2622;
  t3175 = 0.50000000000000000000000000000000e0 * t2626;
  t2460 = 0.56786982094425000000000000000000e-2 * t2620;
  t3146 = t2460 - 0.21751134959804000000000000000000e-1;
  t4091 = t3667 + 0.28801560650267140000000000000000e-2;
  t1815 = -t3961 + 0.28391278634449500000000000000000e0;
  t3966 = t3046 * t2618;
  t4090 = -t3966 + 0.54368101124215626900000000000000e0;
  t2170 = 0.21751134959804000000000000000000e-1 * t2618 - 0.46305794820080000000000000000000e-2;
  t1887 = -0.31228377456598930000000000000000e-2 - t3747;
  t4088 = t1887 * t2604 - 0.23126197987767817000000000000000e-1;
  t4087 = 0.26431758938496000000000000000000e-1 - t2460;
  t3728 = 0.11881704766464000000000000000000e-1 * t2624 + 0.48037471395840000000000000000000e-2 * t2617;
  t1980 = -0.25339016093952000000000000000000e0 - t3728;
  t1896 = 0.2489553776598930000000000000000e-3 + t3747;
  t1853 = t1896 * t2611;
  t4086 = t1853 + 0.53893925569918450000000000000000e0 - t3667;
  t4082 = -0.2e1 * t2619;
  t4081 = -t2605 / 0.2e1;
  t4080 = t2605 / 0.2e1;
  t4079 = t2606 / 0.2e1;
  t2607 = t2621 ^ 2;
  t4078 = -t2607 / 0.2e1;
  t4077 = t2607 / 0.2e1;
  t2608 = t2622 ^ 2;
  t4076 = t2608 / 0.2e1;
  t4075 = t2613 / 0.2e1;
  t2614 = t2628 ^ 2;
  t4074 = -t2614 / 0.2e1;
  t4073 = t2614 / 0.2e1;
  t2615 = t2629 ^ 2;
  t4072 = t2615 / 0.2e1;
  t4071 = -t2618 / 0.2e1;
  t4070 = t2619 / 0.2e1;
  t4069 = -t2620 / 0.2e1;
  t4068 = t2620 / 0.2e1;
  t4067 = -t2621 / 0.2e1;
  t4066 = t2621 / 0.2e1;
  t4065 = -t2622 / 0.2e1;
  t4064 = t2622 / 0.2e1;
  t4063 = t2625 / 0.2e1;
  t4062 = t2626 / 0.2e1;
  t4061 = t2627 / 0.2e1;
  t4060 = -t2628 / 0.2e1;
  t4059 = t2628 / 0.2e1;
  t3288 = 0.9683775114084920000000000000000e-2 * t2617;
  t2203 = -0.11008587194880000000000000000000e-2 - t3288;
  t1746 = t2203 * t2624 + t4282;
  t3714 = -0.25527100084200000000000000000000e-2 * t2624 - 0.10320550495200000000000000000000e-2 * t2617;
  t1992 = -0.54439292389350000000000000000000e-1 + t3714;
  t1554 = t1746 * t2619 + t1992;
  t2108 = 0.48888264403680000000000000000000e-2 * t2624 + 0.19765417918080000000000000000000e-2 * t2617;
  t1961 = t2108 + 0.10425949330324000000000000000000e0;
  t1431 = t1554 * t2620 + t1961;
  t1840 = t1935 - 0.6060977893308120e-2;
  t1690 = t1840 * t2619 - 0.22714792837770000000000000000000e-1 * t2618 + 0.48357317375400000000000000000000e-2;
  t3250 = 0.43502269919608000000000000000000e-1 * t2618;
  t2169 = -0.92611589640160000000000000000000e-2 + t3250;
  t1318 = t1431 * t2625 + t1690 * t2620 + t2169;
  t1907 = t1967 * t2618;
  t1808 = t1907 + 0.10572703575398400000000000000000e0;
  t1733 = t1808 * t2620 - 0.11357396418885000000000000000000e-1;
  t2100 = 0.48888264403680000000000000000000e-2 * t2617 - 0.19765417918080000000000000000000e-2 * t2624;
  t1991 = t2100 - 0.42894239060600000000000000000000e-1;
  t1931 = t1991 * t2619;
  t3744 = -t2249 - t3290;
  t1372 = t2374 + 0.5760312130053428000000000000000e-2 + t3744 - t3319;
  t1899 = -0.4979107553197860000000000000000e-3 + t3744;
  t2470 = 0.27228906756480000000000000000000e-2 * t2624;
  t1977 = -t2470 - t2416 - 0.12085461751057286000000000000000e-1;
  t1988 = 0.22397308370250000000000000000000e-1 - t3727;
  t2380 = 0.96837751140849200000000000000000e-2 * t2610;
  t3307 = t1372 * t2612 + t1899 * t2611 + 0.46660838454822060000000000000000e-2 * t2605 + t1988 * t2619 + t1977 * t2604 + t1980 * t2618 + t2380 + t2248 - 0.10873620224843125380000000000000e1;
  t1143 = t1318 * t2626 + t1733 * t2625 + t1931 - t3961 - 0.25817947234305000000000000000000e-1 + t3307 * t2620;
  t2988 = -t3747 + t4091;
  t1384 = t2988 + t4287;
  t1898 = -0.2489553776598930000000000000000e-3 + t4150;
  t2935 = t2381 - t4090 + t4152 + t4265;
  t2023 = -0.6042730875528643e-2 - t3725;
  t3950 = t2023 * t2604;
  t1157 = t1384 * t2612 + t1898 * t2611 + 0.2333041922741103e-2 * t2605 + t2935 + t3950 + t4375;
  t1695 = -t3402 + t2983;
  t2955 = -t4091 + t4306;
  t1379 = t1695 * t2611 + t2955;
  t3370 = -t3950 + t4233 - t4152;
  t1166 = t1379 * t2612 + t3370 + t4086 - t4375;
  t1288 = (-0.1e1 * t3977 + t1838) * t2620 + t4372;
  t3523 = t4271 - t1538;
  t1180 = t1288 * t2626 + t2620 * t3523 + t3957 + 0.80863245317250000000000000000000e-1;
  t3049 = -0.11198654185125000000000000000000e-1 + t2111;
  t1324 = -t1360 * t2619 + t3049;
  t1976 = -0.37427638925842000000000000000000e-3 + t3717;
  t1502 = t1976 * t2618 + t3155;
  t1183 = t1324 * t2626 + t1502 * t2612 - t1552 * t2625 - t1657;
  t1680 = t2401 + t2986;
  t1517 = t1680 * t2618 + t3046;
  t4041 = t1517 * t2625;
  t1349 = -t3510 + t4041;
  t3309 = t1349 * t2626 + t1559 * t2619 - t4271;
  t1201 = -0.88047764582400000000000000000000e0 + t3309 * t2620;
  t2167 = -t3261 + 0.54457813512960000000000000000000e-2;
  t1671 = -0.96305836223205680000000000000000e-2 * t2610 + t2167 * t2624 + 0.53191491764352000000000000000000e-4 * t2603 + 0.22017174389760000000000000000000e-2 * t2617 + 0.23121910499710648000000000000000e-1;
  t1516 = t1671 * t2618 - t1980;
  t1981 = -0.13379861294270224000000000000000e-1 * t2624 + 0.43868728512658560000000000000000e-2 * t2617 - 0.44088275061402520000000000000000e-1;
  t1346 = t1981 * t2611 + t1516 * t2625 + 0.10572703575398400000000000000000e0 * t2618 + 0.17936986422585684000000000000000e-1 - t2107;
  t3196 = 0.48037471395840000000000000000000e-2 * t2624;
  t3730 = 0.11881704766464000000000000000000e-1 * t2617 - t3196;
  t1550 = t4318 - 0.95593081660407480000000000000000e-1 + t3730;
  t3030 = t2002 * t2619 - 0.22714792837770000000000000000000e-1;
  t1205 = t1346 * t2626 - t3030 * t2625 + t1550 * t2619 + t1992 * t2618 - 0.55505629074184340000000000000000e0;
  t1798 = t1838 * t2619;
  t3850 = t2611 * t2619;
  t1869 = t1967 * t3850;
  t1243 = -t4333 * t2626 + t1869 + t1517 * t3798 - t1798 + 0.3288975154738540e-2;
  t1729 = 0.5004595745882176000000000000000e-2 * t2610 - 0.1256936473410938000000000000000e-2 + t3578;
  t1544 = t1729 * t2619 + t1989;
  t3987 = t1961 * t2618;
  t1606 = -t3957 - t3987 - 0.11683352511943460000000000000000e1;
  t3185 = 0.43502269919608000000000000000000e-1 * t2625;
  t1752 = -t3185 + t3987 + 0.20699436005309600000000000000000e0;
  t1758 = -t1798 + 0.3288975154738540000000000000000e-2;
  t1816 = t1931 - 0.12056561435880000000000000000000e0;
  t1826 = t3966 - 0.4741755542971769000000000000000e-2;
  t3170 = 0.56786982094425000000000000000000e-2 * t2627;
  t3058 = t2625 * t3170;
  t3805 = t2622 * t2629;
  t3610 = t3805 / 0.2e1;
  t3648 = t2621 * t3790;
  t3821 = t2620 * t2627;
  t3708 = -0.2e1 * t3821;
  t3812 = t2621 * t2628;
  t3986 = t1961 * t2625;
  t1017 = ((t1166 * t3708 + (t3523 + t4374) * t2613 - t1180 * t2620 + (0.10572703575398400000000000000000e0 * t2620 - 0.11357396418885000000000000000000e-1) * t3786 + 0.2e1 * t1826 * t3821 + t1815 * t2627) * t2614 + (-t1183 * t2620 + ((-t1557 - t3972) * t2626 + t1758 + (t3977 + t4044) * t2619) * t2627) * t3812 - t1752 * t2620 + (t2169 + t3986) * t3790 + t1816 * t2627) * t4076 + ((t1205 * t3708 + ((t1554 * t2625 + t1690) * t2626 + t1808 * t2625 + t3307) * t2613 - t1143 * t2620 - t1755 * t3790 + (t3185 + t1606) * t2627) * t2628 - t1243 * t3817 + (t2619 * t3319 + t1544) * t3648 + t2621 * t1552 * t3786 + t4236 * t3813) * t3610 + (-0.1e1 * t1201 * t2620 + (-0.2e1 * t1157 * t2620 + 0.18916511922000000000000000000000e0 + t3309 * t2627) * t2627) * t4072 + (-t1726 - t3957 + 0.79961440050675000000000000000000e0) * t4069 + t3058 + (t3961 - 0.47307790556449500000000000000000e0) * t4061;
  t2637 = q_state_dot(1);
  t4057 = t1017 * t2637;
  t1283 = (t1544 + (-0.1e1 * t3694 - t4025) * t2619) * t2620 + t1991;
  t3959 = t3047 * t2620;
  t1417 = t1513 - t3959;
  t1292 = t1417 * t2625 + t2171 * t2620 - t3510;
  t3479 = -0.1e1 * t3972 - t1557;
  t1364 = t2620 * t3479 + t1989;
  t1661 = t1694 * t2611;
  t3768 = t1661 - t3667;
  t1385 = -0.4533121716787550000000000000000e-3 + t3401 + t3748 + t3768;
  t1685 = t1961 * t2620 + t3047;
  t1460 = t1685 * t2625 + t2169 * t2620 - t2171;
  t1490 = t2612 * t1506;
  t1702 = t1748 * t3793;
  t3649 = t2621 * t3791;
  t3474 = t2619 * t3649;
  t3663 = t2618 * t3798;
  t3476 = t1968 * t3663;
  t3657 = t2619 * t3791;
  t3526 = -0.2e1 * t3657;
  t3642 = t2621 * t3793;
  t3647 = t2621 * t3783;
  t3650 = t2620 * t3790;
  t3848 = t2611 * t2626;
  t3703 = t1694 * t3848;
  t3814 = t2612 * t2621;
  t3815 = t2621 * t2626;
  t3853 = t2605 * t1506;
  t1019 = ((t1490 - 0.1e1 * t3853 + (-0.1e1 * t2613 + t2627) * t3956) * t2614 + t3956 + ((0.1e1 * t4376 - 0.1e1 * t1288 * t2627) * t2614 + (-0.1e1 * t1324 * t2627 - 0.1e1 * t1364) * t3812 - 0.1e1 * t1460) * t2619 + (((0.1e1 * t3958 - 0.1e1 * t2171) * t2627 - t4372) * t3812 + (t1506 * t2613 * t2614 - t1360 * t3647) * t2626 + (((-0.2e1 * t1379 - 0.46660838454822060000000000000000e-2) * t2613 - 0.2e1 * t1385 + 0.6595987621373214e-2) * t2614 - 0.2e1 * t1502 * t3647) * t2619 + (t3479 * t2627 * t2614 + (t3977 - 0.1e1 * t1838) * t3812 + t1991) * t2620) * t2626) * t4076 + (((-0.1e1 * t1346 * t2619 + (t1550 - 0.1e1 * t3953) * t2626) * t2613 + (t1372 * t3526 + (t1746 * t2625 + t1840) * t4189 - 0.1e1 * t1318 * t2619 + (0.93321676909644120000000000000000e-2 * t2619 + t1988) * t3791 + t1991 * t2626) * t2627 - 0.1e1 * t1292 * t2619 + t1973 * t3793 - 0.1e1 * t1989 * t3791 + t1557 * t2626) * t2628 + (0.1e1 * t4333 * t2619 + (-0.1e1 * t3510 + t4041) * t2626) * t3813 + 0.2e1 * t1507 * t3474 + (t1729 + t3319) * t2620 * t3814 - 0.1e1 * t1283 * t3818 + (-0.1e1 * t1961 - t3959) * t3642 + t2171 * t3649 - 0.1e1 * t2169 * t3815) * t3610 + (((t1810 * t2626 - t1702) * t2626 + t3956) * t2613 + t4333 * t3650 + t3711 * t1507 + (-0.1e1 * t4376 - 0.1e1 * t1349 * t3821 + ((-0.2e1 * t1384 + 0.4666083845482206e-2) * t2613 - 0.2e1 * t1360) * t2626) * t2619) * t4072 + (-0.1e1 * t3956 + t4339) * t4061 + t2619 * t3703 - 0.1e1 * t2626 * t3476 + (-0.36699518879455040000000000000000e-2 + 0.1e1 * t3747) * t3826 - (t4081 + t4094) * t1506;
  t4056 = t1019 * t2637;
  t3710 = -0.2e1 * t3832;
  t1378 = t1696 * t3710 + t3508 + 0.6245675491319786e-2 * t3832;
  t3702 = t1694 * t3832;
  t1404 = -t3508 - 0.2e1 * t3702;
  t1425 = t1552 * t2620 - t1961 * t2619;
  t1508 = t4350 * t3826;
  t3235 = 0.11357396418885000000000000000000e-1 * t2620;
  t1730 = t1907 + 0.52863517876992000000000000000000e-1 * t2606 - t3235;
  t1751 = -t1813 + 0.43502269919608000000000000000000e-1 * t2620;
  t3688 = t2023 * t3832;
  t1880 = 0.2e1 * t3688;
  t1881 = -0.2e1 * t3688;
  t3083 = 0.62456754913197860000000000000000e-2 * t3832;
  t3404 = -t3083 - t3508;
  t3643 = t2619 * t3797;
  t3475 = t2618 * t3643;
  t3411 = -0.2e1 * t3475;
  t3527 = t2620 * t3710;
  t3761 = -0.2e1 * t3694 - t3184;
  t3587 = t3761 + t1643;
  t3602 = t3790 / 0.2e1;
  t3608 = -t3797 / 0.2e1;
  t3620 = t3826 / 0.2e1;
  t3673 = t2612 * t3817;
  t3675 = t2611 * t3823;
  t3849 = t2611 * t2620;
  t3695 = t1967 * t3849;
  t3700 = t1896 * t3832;
  t3712 = t2604 - 0.1e1 * t2611;
  t3965 = t3046 * t2625;
  t3759 = t3851 + t3965;
  t3766 = t1748 * t3798 - t3958;
  t3819 = t2621 * t2618;
  t3976 = t1967 * t2625;
  t3978 = t1967 * t2604;
  t4026 = t1680 * t2611;
  t1020 = ((((t1695 * t3710 + t3404) * t2612 + (t4369 - t4229) * t2626 - 0.2e1 * t3700 + t1881 - t3508) * t2613 + ((0.1e1 * t1418 * t2618 - t2509) * t2626 + (-t1663 * t3848 - 0.1e1 * t4296 + t3958 + ((0.52863517876992000000000000000000e-1 + 0.2e1 * t1907) * t2626 - t4010) * t2625) * t2620) * t2627 + t1404 * t2612 - t1508 - t1663 * t3710 + t3977 - t1730 * t2618 + t2606 * t3965 - t3047 * t3797) * t2614 + (((t1976 * t2625 + t4318) * t2612 + (t1869 + (-0.1e1 * t3978 + t4366) * t2619) * t2626 + t1552 * t2618 - t4149) * t2627 + (t3973 - t4346) * t3791 + t1967 * t3411 + t1663 * t3675 - t1418 * t3835 - t3184 * t3823 + t2304) * t3812 + (t3250 + t3986) * t2627 + (-t1685 * t2618 + t2620 * t3185 - t2509) * t2626) * t4076 + ((((t1671 * t2611 - 0.1e1 * t1516 * t2618) * t2626 + t3030 * t2618 + ((-0.2e1 * t1981 * t2618 + 0.10572703575398400000000000000000e0) * t2626 + t1742 * t2619 + t1992) * t2625) * t2613 + ((t3977 - 0.1e1 * t3978 - t4367) * t4189 + (-t1431 * t2618 + t3030 * t3797 + t3185) * t2626 + t1899 * t3527 + t3695 - t1733 * t2618 + (t1977 * t4083 + t1980) * t3797 - t3958) * t2627 + (-t1417 * t2618 + t2509 * t2620 + t3587) * t2626 - t1751 * t2618 - t1961 * t3797 + t3766) * t2628 + ((t1749 * t2625 + t3973) * t2626 + (t4026 - t3184 + (-0.2e1 * t3976 - 0.1e1 * t1517) * t2618) * t2619) * t3813 + t4329 * t3673 + (t1967 * t3712 + t4367) * t3474 - t1425 * t3819 + t4149 * t3817 - t3185 * t3818) * t3610 + ((t1378 * t2612 + t4229 * t2626 + t1880 + (-t1556 * t2626 - 0.2e1 * t1898 * t2625 - t1809) * t2618 + t3759) * t2613 + ((-t1517 * t2618 + t3761 + t4026) * t2626 + t4296 - t1749 * t3798 - t3958) * t3821 + (-t3977 + t3978 - t4366) * t2612 - t4329 * t3826 + t1378) * t4072 - t4217 * t3602 + t4350 * t3620 - t2605 * t3702 + t3851 * t4081 + (-t2605 * t3975 + t3235 - 0.52863517876992000000000000000000e-1) * t4071 - t3047 * t3608 - t3965 / 0.2e1;
  t4055 = t1020 * t2637;
  t1073 = 0.72089127222315021200000000000000e0 + t1205 * t2613 + t1143 * t2627 + t1292 * t2626 + t1751 * t2625 + t1606 * t2620 + t1538 - t3961;
  t1468 = t1506 * t3826;
  t1074 = -0.62236259692023701500000000000000e0 + t1166 * t2613 + t1180 * t2627 + t1385 * t2612 + t1468 - t1643 + t1730 * t2625 + t1826 * t2606 + t1815 * t2620 + 0.3297993810686607e-2 * t2605 - t3402 + t3581;
  t1108 = t1183 * t2627 + t1364 * t2626 + t1758 * t2620 + t2075 + 0.243824841901488000000000000000e-3 + (t3695 + t4046) * t2619;
  t2809 = t1243 * t2627 + t1283 * t2626 + t1425 * t2625 - 0.26594038206575168000000000000000e-1 - 0.1e1 * t2169 * t2619;
  t3071 = 0.50000000000000000000000000000000e0 * t3805;
  t1021 = -t1073 * t2621 * t3071 + 0.50000000000000000000000000000000e0 * (-0.1e1 * t2607 + t2614) * t2608 * t1108 + (-0.10000000000000000000000000000000e1 * t1074 * t2621 * t2608 + (-t1507 * t4189 + t1657 * t2620 + t2809) * t3071) * t2628;
  t4054 = t1021 * t2637;
  t1511 = t1524 * t3826;
  t3193 = 0.63217394930520320000000000000000e-2 * t2624;
  t3923 = t2107 * t2618;
  t1534 = (t2380 - t2470 + (t3193 - 0.1e1 * t2155) * t2617) * t2625 + t3923;
  t3740 = -t2617 * t3193 + t2470;
  t1711 = t2155 * t2617 - t2380 + t3740;
  t1822 = t1858 * t2612;
  t3122 = t2624 * t3289;
  t1865 = -t2390 + t3122 + t3279;
  t3215 = 0.27521467987200000000000000000000e-3 * t2624;
  t3687 = t2111 * t3834;
  t3466 = t3687 / 0.2e1;
  t2918 = t3215 + t3466;
  t3456 = t3739 + t4219;
  t3907 = t3729 * t2618;
  t2976 = t1414 * t2612 + t3456 + t3907 + t4145 - t4365;
  t3192 = 0.19367550228169840000000000000000e-1 * t2624;
  t3919 = t4130 * t2625;
  t3501 = -t3718 + t3919;
  t3575 = t2624 * t3288 + t3732;
  t3588 = -t1998 - t4356;
  t3625 = t3832 / 0.2e1;
  t3686 = t2111 * t3793;
  t3757 = -t3686 - t3916;
  t3796 = t2625 * t2621;
  t3881 = t2200 * t2617;
  t3920 = t2111 * t2625;
  t1025 = ((t4112 * t2613 + ((-t2620 * t4359 + t3920) * t2626 + t4130 * t3643 + t4356 * t2620 + t3916) * t2627 + t1406 + t1511 + t2606 * t3907 - t3687 + t1710 - t3317) * t2614 + ((t1534 * t2612 - t3723 * t2626 + ((t1672 + 0.1e1 * t2001 + t1856) * t2626 + t3920) * t2619 - t1524) * t2627 + ((-t4342 + t3919) * t2620 + t3723) * t2626 + t3717 * t3675 + (-t2620 * t4326 - t2111) * t3798 + t2102 * t3823) * t3812 - t2100 * t3787 + (-t2100 * t2620 + t2111) * t3793 + t2108 * t3823 + t3916) * t4076 + (((((0.13379861294270224000000000000000e-1 * t2617 + 0.43868728512658560000000000000000e-2 * t2624) * t2611 + ((-t2383 + 0.22017174389760000000000000000000e-2 * t2624) * t2618 + t3196 + ((t3192 - 0.1e1 * t2167) * t2618 - 0.11881704766464000000000000000000e-1) * t2617) * t2625 + t3717) * t2626 + t2107 * t3798 + (t1711 * t2618 + t3728) * t2619 + t3727 * t2618) * t2613 + (-t2100 * t3793 + t2108 * t2619 - t2033 + ((t3575 - t3317) * t2612 + ((-0.9683775114084920000000000000000e-2 * t2610 - 0.1e1 * t2203 * t2617 + t3740) * t2619 + t3727) * t3793 + t3575 * t2611 + t3714 * t2619 + (t2408 - t3208) * t2604 - t2617 * t3192 + t2383 - 0.31608697465260160000000000000000e-2 * t2603 + (-0.1e1 * t2107 * t3826 + t3717 * t2625 + t3730) * t2618) * t2620) * t2627 + ((-t2111 * t2620 - t4326) * t2625 + t2822) * t2626 + (t2100 * t2618 - t3916) * t2620 + t3588) * t2628 + (((t3881 + t4307) * t2618 + t3501) * t2626 + (0.1e1 * t2036 - t4035 + t2102) * t2619) * t3813 + (t1711 * t2625 - t3923) * t3673 + (((-0.1e1 * t1856 + t3317) * t2619 + t3723) * t2620 + t2108) * t3815 + ((-t2111 * t2619 + t1706) * t2620 + t2100 * t2619) * t3796 + t3817 * t4241) * t3610 + ((t1865 * t2611 + t2976) * t2613 + (t1392 - t2033 + (-0.1e1 * t3919 + (-0.1e1 * t3881 - t4307) * t2618 + t3718) * t2619) * t3821 + (-t2363 + t3317 + t3739) * t2612 + t1534 * t3826 + t1414) * t4072 + t3757 * t4061 + t1822 / 0.2e1 - t1524 * t3620 + t1678 * t4080 + t2102 * t2605 * t3625 - t3907 / 0.2e1 - t2419 + t2918;
  t4053 = t1025 * t2637;
  t1371 = t2988 + t4167;
  t2925 = 0.3030488946654060e-2 * t2619 - 0.24178658687700000000000000000000e-2;
  t1373 = -t2925 - t4370;
  t1963 = -0.60427308755286430000000000000000e-2 - t3725;
  t1906 = t1963 * t2604;
  t1155 = t1371 * t2612 + t1373 * t2626 - t1853 + t1906 + t2378 + t2935;
  t4051 = t1155 * t2620;
  t1665 = -t2367 + t2984;
  t1514 = t1665 * t2618 + t1978;
  t4043 = t1514 * t2625;
  t4040 = t1519 * t2612;
  t4027 = t1665 * t2611;
  t2017 = t3152 + t3402;
  t1697 = t2017 + t4232;
  t4024 = t1697 * t2618;
  t1673 = t1705 * t2618;
  t3905 = t2122 * t2628;
  t1715 = t3905 + t4294;
  t4019 = t1715 * t2623;
  t4018 = t1715 * t2630;
  t4013 = t1744 * t2627;
  t4008 = t1753 * t2627;
  t4000 = t1855 * t2611;
  t3996 = t1882 * t2625;
  t1883 = -t2246 + 0.34240000000000000000000000000000e-2 * t2610 + 0.29200000000000000000000000000000e-2;
  t3995 = t1883 * t2618;
  t3994 = t1883 * t2625;
  t3993 = t1884 * t2604;
  t1945 = 0.3122837745659893e-2 + t3747;
  t3988 = t1945 * t2604;
  t1904 = t1962 * t2625;
  t3984 = t1962 * t2627;
  t3981 = t3050 * t2627;
  t3974 = t1970 * t2620;
  t1972 = t2474 - t2158;
  t1909 = t1972 * t2627;
  t3970 = t3044 * t2620;
  t3969 = t1978 * t2619;
  t3968 = t1978 * t2620;
  t1918 = t1978 * t2627;
  t2174 = -t3170 + 0.56786982094425000000000000000000e-2;
  t3232 = 0.26431758938496000000000000000000e-1 * t2620;
  t1983 = t2174 - t3232;
  t3967 = t1983 * t2618;
  t3964 = t1986 * t2620;
  t3963 = t1986 * t2621;
  t3962 = t1986 * t2626;
  t1932 = t1986 * t2627;
  t1990 = 0.21800000000000000000000000000000e-3 + t3720;
  t3955 = t1990 * t2604;
  t3954 = t1990 * t2611;
  t2003 = -t3719 + 0.9356909731460500000000000000000e-4;
  t3952 = t2003 * t2619;
  t3951 = t2003 * t2625;
  t3947 = t2025 * t2618;
  t1960 = t2025 * t2625;
  t3946 = t2025 * t2628;
  t3940 = t2875 * t2621;
  t3939 = t2062 * t2618;
  t3936 = t2064 * t2618;
  t3926 = (0.26595745882176e-4 * t3838 + t2479) * t2618;
  t3198 = 0.29640000000000000000000000000000e-2 * t2624;
  t3259 = 0.47840000000000000000000000000000e-2 * t2617;
  t2101 = t3198 + t3259;
  t3925 = t2101 * t2611;
  t3924 = t4222 * t2627;
  t3922 = t3719 * t2626;
  t3921 = t3720 * t2625;
  t3918 = t2114 * t2627;
  t3917 = t2115 * t2625;
  t2030 = t3724 * t2627;
  t3914 = t2852 * t2619;
  t3912 = t2852 * t2626;
  t3911 = t2852 * t2628;
  t2040 = t2119 * t2620;
  t3910 = t2119 * t2625;
  t3167 = 0.24444132201840000000000000000000e-2 * t2628;
  t2126 = -t3167 - t2464;
  t3904 = t2126 * t2624;
  t2152 = t2521 * t2619;
  t3903 = t2152 * t2621;
  t3900 = t2157 * t2618;
  t3891 = t2165 * t2620;
  t3890 = t2170 * t2620;
  t3889 = t2170 * t2621;
  t3888 = t2170 * t2628;
  t3253 = 0.56786982094425000000000000000000e-2 * t2618;
  t2172 = -0.12089329343850000000000000000000e-2 + t3253;
  t3887 = t2172 * t2621;
  t3886 = t2172 * t2626;
  t2076 = t2172 * t2628;
  t2177 = 0.12669508046976000000000000000000e0 + t3262;
  t3885 = t2177 * t2625;
  t2079 = t4089 * t2620;
  t3884 = t2179 * t2619;
  t3883 = t2883 * t2628;
  t3882 = t2182 * t2621;
  t2083 = t2182 * t2628;
  t3880 = t2201 * t2618;
  t2084 = t2201 * t2621;
  t3879 = t2201 * t2628;
  t3878 = t2205 * t2627;
  t2236 = 0.93569097314605e-4 + t3264;
  t3876 = t2236 * t2618;
  t2362 = -0.316e0 * t2627 + t3572 - 0.384e0;
  t3868 = t2362 * t2625;
  t3866 = t2523 * t2630;
  t3860 = t2527 * t2619;
  t3855 = t2604 * t2620;
  t3854 = t2605 * t1480;
  t3852 = t2605 * t2621;
  t3847 = t2611 * t2627;
  t1528 = -t3934 - t3720 - 0.8292e-2 + t3669;
  t1337 = 0.15592e-1 + t1528 * t2626 + t4240;
  t3844 = t2613 * t1337;
  t3843 = t2613 * t2621;
  t3842 = t2613 * t2628;
  t3841 = t2613 * t2629;
  t3840 = t2617 * t2618;
  t3839 = t2617 * t2619;
  t3837 = t2617 * t2629;
  t3836 = t2618 * t2003;
  t3833 = t2618 * t2622;
  t3831 = t2618 * t2626;
  t3830 = t2618 * t2628;
  t3829 = t2618 * t2629;
  t3827 = t2619 * t2624;
  t3825 = t2619 * t2627;
  t3824 = t2619 * t2629;
  t3816 = t2621 * t2624;
  t3811 = t2622 * t2614;
  t3807 = t2622 * t2627;
  t3804 = t2623 * t2621;
  t3803 = t2623 * t2622;
  t3802 = t2623 * t2628;
  t3801 = t2623 * t2629;
  t3799 = t2624 * t2629;
  t3795 = t2625 * t2622;
  t3794 = t2625 * t2624;
  t3792 = t2625 * t2628;
  t2970 = t2628 * t2522;
  t3785 = t2628 * t2619;
  t3781 = t2629 * t2621;
  t3779 = t2629 * t2627;
  t3778 = t2629 * t2628;
  t3777 = t2630 * t2621;
  t3776 = t2630 * t2622;
  t3775 = t2630 * t2628;
  t3774 = t2630 * t2629;
  t2271 = t2618 * t2471;
  t1622 = t2271 + t4161;
  t3773 = t1622 * t3826 + t4295;
  t1481 = t3763 - t4268;
  t3772 = t1481 * t2612 - t1581;
  t3670 = t1884 * t3832;
  t3407 = 0.2e1 * t3670 + t3503;
  t3771 = t2612 * t3407 + t4321;
  t3770 = t1694 * t3787 + t1918;
  t1667 = t1956 + t4232;
  t1641 = t1667 * t2611;
  t3769 = t1641 + 0.2e1 * t3667;
  t2080 = t4089 * t2627;
  t2302 = t2627 * t2478;
  t3756 = t2080 + t2302;
  t2240 = t2621 * t2407;
  t2293 = t2621 * t2474;
  t3755 = t2240 - t2293;
  t2292 = t2621 * t3211;
  t3227 = 0.24444132201840000000000000000000e-2 * t2621;
  t3754 = t2617 * t3227 - t2292;
  t2286 = t2621 * t2469;
  t3753 = t2414 * t2621 + t2286;
  t2294 = t2621 * t3203;
  t3752 = t2464 * t2617 - t2294;
  t3751 = t3724 * t2621;
  t2288 = t2621 * t3216;
  t3750 = -t2617 * t3230 + t2288;
  t3737 = -t2162 * t3794 - t2386 * t2625;
  t3568 = 0.825e-1 * t2629;
  t2552 = t2621 * t3568;
  t3444 = t2627 * t3568;
  t3736 = -t2621 * t3444 + t2552;
  t2549 = t2622 * t3570;
  t3569 = 0.825e-1 * t2628;
  t3446 = t2620 * t3569;
  t3735 = -t2629 * t3446 + t2549;
  t3168 = 0.26431758938496000000000000000000e-1 * t2627;
  t3716 = t2460 - t3168;
  t3707 = -0.2e1 * t3832;
  t3706 = -0.2e1 * t3826;
  t3704 = t4220 * t3783;
  t3699 = t1945 * t3855;
  t3698 = t1945 * t3784;
  t3693 = t1968 * t3834;
  t3692 = t1968 * t3791;
  t3691 = t2621 * t3851;
  t1871 = t1968 * t3787;
  t3690 = t2628 * t3851;
  t3684 = t2625 * t3898;
  t3680 = t2522 * t3782;
  t3679 = t2522 * t3810;
  t3678 = t3123 * t3833;
  t3676 = t2604 * t3823;
  t3674 = t2611 * t3785;
  t3672 = t2612 * t3782;
  t3671 = t1855 * t3832;
  t3668 = t1968 * t3819;
  t3662 = t2618 * t3786;
  t3661 = t2618 * t3782;
  t3660 = t1480 * t3826;
  t3659 = t2098 * t3798;
  t3658 = t2106 * t3850;
  t3655 = t2619 * t3783;
  t3654 = t1858 * t3855;
  t3653 = t2620 * t3803;
  t3652 = t2620 * t3776;
  t3651 = t2623 * t3784;
  t3646 = t2619 * t3809;
  t3645 = t2620 * t3804;
  t3644 = t2623 * t3783;
  t3641 = t2620 * t3780;
  t3640 = t2626 * t3783;
  t3639 = t2626 * t3782;
  t3637 = t2618 * t3783;
  t3634 = t2620 * t3779;
  t3633 = t2620 * t3777;
  t3632 = t4320 / 0.2e1;
  t3631 = -t1858 * t2604 / 0.2e1;
  t3630 = t2606 * t4058;
  t3629 = t3847 / 0.2e1;
  t3627 = t3841 / 0.2e1;
  t3626 = t3837 / 0.2e1;
  t3624 = -t3830 / 0.2e1;
  t3623 = -t3829 / 0.2e1;
  t3622 = t3829 / 0.2e1;
  t3621 = -t3828 / 0.2e1;
  t3619 = -t3825 / 0.2e1;
  t3618 = t3825 / 0.2e1;
  t3617 = t3824 / 0.2e1;
  t3616 = -t3818 / 0.2e1;
  t3615 = t3812 / 0.2e1;
  t3614 = t3811 / 0.2e1;
  t3613 = -t3810 / 0.2e1;
  t3612 = -t3808 / 0.2e1;
  t3611 = -t3807 / 0.2e1;
  t3609 = t3799 / 0.2e1;
  t3607 = t3797 / 0.2e1;
  t3606 = -t3795 / 0.2e1;
  t3605 = -t3793 / 0.2e1;
  t3603 = t3792 / 0.2e1;
  t3601 = t3789 / 0.2e1;
  t3600 = -t3788 / 0.2e1;
  t3599 = t3788 / 0.2e1;
  t3598 = t3785 / 0.2e1;
  t3597 = -t3784 / 0.2e1;
  t3595 = t3783 / 0.2e1;
  t3594 = -t3782 / 0.2e1;
  t3593 = t3782 / 0.2e1;
  t3592 = t3781 / 0.2e1;
  t3591 = t3780 / 0.2e1;
  t3590 = t3779 / 0.2e1;
  t3586 = t1673 - t2103;
  t2517 = 0.21751134959804000000000000000000e-1 * t2628;
  t3097 = t2621 * t2390;
  t3584 = t2159 * t3816 + t2517 - t3097;
  t3583 = t2027 + t3719;
  t3580 = t4210 * t2621;
  t1656 = t2159 * t3794 - t2625 * t4133;
  t3567 = 0.384e0 * t2629;
  t3574 = -t3567 * t3817 + t3736;
  t3564 = 0.5317e-1 * t2622;
  t3562 = 0.5317e-1 * t2629;
  t3561 = 0.3495e-2 * t2630;
  t2339 = -0.341e-3 - t3267;
  t3560 = t2339 * t2618 + 0.3449e-2;
  t3554 = 0.61597e-1 * t2620;
  t3545 = 0.61597e-1 * t2627;
  t3543 = 0.735522e0 * t1160;
  t3541 = 0.735522e0 * t2618;
  t3540 = 0.735522e0 * t2620;
  t3539 = 0.104419e0 * t2622;
  t3536 = 0.646926e0 * t2623;
  t3535 = 0.735522e0 * t2625;
  t3534 = 0.735522e0 * t2626;
  t3531 = 0.735522e0 * t2627;
  t1362 = t3667 + t4167 - t4330;
  t3525 = t1362 * t2619 + t3044;
  t3073 = t2621 * t3199;
  t1634 = -t3073 + t3882 + t3946;
  t2287 = t2621 * t3206;
  t2163 = 0.27219646194675000000000000000000e-1 + t3271;
  t3504 = t2163 + t3984;
  t1377 = t1634 * t2620 + t2621 * t3504 + t2287;
  t2234 = 0.4841887557042460e-2 * t2617 + 0.55042935974400000000000000000000e-3;
  t2931 = t2234 * t2624 + t3020;
  t3477 = t1968 * t3637;
  t1493 = -0.1e1 * t3477 + t2931 * t2621;
  t3524 = t1493 * t2619 + t1377;
  t3522 = t1531 + t1960;
  t3520 = t1725 - 0.82500000000000000000000000000000e-1 + t4352;
  t1832 = t2274 + t3302;
  t3514 = t1832 - t4346;
  t1833 = -t3203 + t3151 - t2451;
  t3511 = t1833 + t3851;
  t1844 = t2159 * t2628 + t2626 * t3230;
  t2314 = t2628 * t2390;
  t3509 = t1844 * t2624 - t2314;
  t2078 = t2172 * t2627;
  t3507 = t2625 * t3984 - t2078;
  t3506 = t1972 * t2620 - t1914;
  t3500 = -t2883 + t3897;
  t3490 = 0.1632768e-2 * t2620;
  t3489 = 0.4038528e-2 * t2620;
  t3488 = 0.1225946e1 * t2623;
  t3487 = 0.1666555e1 * t2623;
  t3486 = 0.3587895e1 * t2623;
  t3485 = 0.1225946e1 * t2630;
  t3484 = 0.1666555e1 * t2630;
  t3483 = 0.3228604e1 * t2630;
  t3482 = 0.3587895e1 * t2630;
  t3480 = -t3719 - 0.1e1 * t2027;
  t3478 = t1945 * t3662;
  t3473 = t2628 * t3657;
  t3472 = t2619 * t3639;
  t3470 = t2621 * t3634;
  t3469 = t2627 * t3631;
  t3468 = -t3699 / 0.2e1;
  t3467 = t1968 * t3629;
  t3464 = t2612 * t3593;
  t3463 = -t1744 * t3834 / 0.2e1;
  t3462 = t2613 * t3592;
  t3461 = t2625 * t3618;
  t3460 = t2620 * t3591;
  t3459 = t2618 * t3617;
  t3458 = t2629 * t3616;
  t3457 = t2626 * t3592;
  t3455 = t3567 * t3783 + t3735 + 0.384e0 * t3810;
  t3454 = 0.3127439544e-2 * t2568;
  t3450 = 0.3127439544e-2 * t2624;
  t3448 = 0.3127439544e-2 * t2626;
  t3447 = 0.7735484874e-2 * t2626;
  t3445 = t2622 * t3571;
  t3443 = -0.1e1 * t4317 - 0.1e1 * t1972;
  t3442 = 0.275214679872e-3 * t2625;
  t3441 = 0.680722668912e-3 * t2625;
  t3440 = t2626 * t3545;
  t3437 = 0.2580137623800e-3 * t2618;
  t3436 = 0.6381775021050e-3 * t2618;
  t3435 = 0.2580137623800e-3 * t2620;
  t3433 = 0.2580137623800e-3 * t2621;
  t3432 = 0.6381775021050e-3 * t2621;
  t3431 = 0.2444413220184e-2 * t2621;
  t3430 = 0.2580137623800e-3 * t2625;
  t3429 = 0.6381775021050e-3 * t2625;
  t3428 = 0.2580137623800e-3 * t2627;
  t3425 = 0.2970426191616e-2 * t2627;
  t3424 = 0.2580137623800e-3 * t2628;
  t3423 = 0.6381775021050e-3 * t2628;
  t2060 = t2361 * t3558 + 0.374176e-3 * t2620;
  t3419 = t2060 * t3535;
  t2066 = -t2361 * t3566 + 0.925496e-3 * t2620;
  t3418 = t2066 * t3535;
  t3415 = t2621 * t3540;
  t3414 = t2628 * t3540;
  t3412 = t2625 * t3534;
  t3409 = t2003 * t3825 - t3693;
  t1268 = t1481 * t3709 + t1618 * t2605 - t1599;
  t1803 = -0.2e1 * t3670;
  t1512 = t1803 - t3503;
  t3403 = t2083 - t2084 + t3904;
  t1777 = t4278 + 0.316e0;
  t1389 = t1777 * t2629 + t4237;
  t3397 = t1389 * t3484;
  t1790 = t2355 * t2629 - t4260;
  t3391 = t1790 * t3482;
  t3389 = t4281 * t3483;
  t3388 = t2619 * t3490;
  t3387 = t2619 * t3489;
  t3383 = 0.1096718212816464e-2 * t2624;
  t2275 = t2618 * t3214;
  t3382 = t2275 + 0.2390110552949070e-2;
  t2881 = -0.21447119530300000000000000000000e-1 + t2410;
  t3024 = -t2881 + t3211;
  t1577 = -0.1e1 * t1833 * t2628 + t3024 * t2621;
  t3381 = -0.1e1 * t3690 + t1577;
  t3380 = t2621 * t1514;
  t1522 = t2618 * t4210 + t4205;
  t3377 = (t1522 - t4247) * t2627;
  t3373 = t2618 * t3458;
  t3372 = t2619 * t3460;
  t3371 = t3470 / 0.2e1;
  t1611 = -0.1e1 * t3938 + 0.458e-3 - t3991;
  t2335 = 0.8292e-2 - t3266;
  t2839 = -0.1e1 * t3934 + t3669 - t2471 - 0.1e1 * t2335;
  t2766 = t1611 * t2626 + t2619 * t2839 - 0.17282e-1;
  t2334 = t3259 + 0.1364e-2;
  t3002 = -t3198 - 0.1e1 * t2334;
  t1614 = -0.1e1 * t3994 + 0.8468e-2 + t3002 * t2618;
  t2923 = t1614 * t2612 - t4327;
  t1169 = 0.95220000000000000000000000000000e-2 + t2923 * t2627 + t2766 * t2620;
  t1527 = t3937 - t2115 + 0.4146e-2 - t3670;
  t1736 = t2623 * t2871 - t3866;
  t2749 = t3772 + t4305;
  t2908 = 0.31784000000000000000000000000000e-1 - t2018 + t3762 + t3772;
  t2715 = t1337 * t3821 + t2613 * t2749 + t2908;
  t2713 = t2622 * t2715;
  t2336 = 0.4146e-2 - t3270;
  t2840 = -0.1e1 * t3937 + t3670 - t3207 - 0.1e1 * t2336;
  t2767 = t1609 * t2626 + t2619 * t2840 - 0.8641e-2;
  t2755 = t2629 * t2767;
  t1462 = t1480 * t2612;
  t2860 = t1462 - t4305 + t1581;
  t2818 = t2629 * t2860;
  t2803 = -t2818 / 0.2e1;
  t2927 = t2620 * t3560 - 0.12805000000000000000000000000000e-1;
  t2943 = -t2970 - t4294;
  t3142 = -t2571 - 0.1e1 * t3870;
  t2977 = 0.825e-1 + t3142;
  t3068 = t2629 * t3213;
  t2994 = t2620 * t3068;
  t3034 = -0.19192000000000000000000000000000e-1 + t1827 * t2619;
  t3281 = 0.17939475000000000000000000000000e1 * t1790;
  t3099 = t2630 * t3281;
  t3100 = t2623 * t3281;
  t3220 = 0.61297300000000000000000000000000e0 * t2623;
  t3103 = t1578 * t3220;
  t3104 = t1389 * t3158;
  t3105 = t1389 * t3218;
  t1369 = t1572 * t2623 + t4018;
  t3106 = t1369 * t3160;
  t1732 = -t2004 + t3906;
  t1520 = t1732 * t2629 - t2356 * t3810 + t2622 * t3532 + t2599;
  t1354 = t1520 * t2630 + t4019;
  t3107 = t1354 * t3220;
  t1367 = t4008 + 0.31600000000000000000000000000000e0 - t4353;
  t3041 = -t2621 * t4220 + t2628 * t3520;
  t1192 = t1367 * t2629 + t2622 * t3041;
  t3111 = t1192 * t3161;
  t3113 = t1192 * t3221;
  t2646 = -0.1e1 * ((-0.1e1 * (-0.1e1 * t4312 + 0.825e-1 - 0.1e1 * t2226) * t2621 - 0.1e1 * t2841) * t3774 + t4341 * t2623) * t3105 - 0.1e1 * (t2630 * t4341 + t3801 * t4117) * t3104 + (t2088 * t2623 + t2629 * t3116) * t3100 - 0.1e1 * ((-0.1e1 * t4003 + (-0.1e1 * t4029 - 0.1e1 * t1714) * t2621) * t3801 + (-0.1e1 * t4290 + (t3359 - 0.825e-1) * t2628) * t2630) * t3111 + t1169 * t2621 * t3806 + (-0.1e1 * t2618 * t2994 + t2621 * t2713 + t2627 * t2755 + t2629 * t2927) * t4066 - 0.1e1 * ((t4028 + (-0.1e1 * t4004 - 0.1e1 * t4106) * t2621) * t3774 - 0.1e1 * t1775 * t3644 - 0.1e1 * t1648 * t3804 + t4105 * t3651 - 0.1e1 * t2623 * t3569) * t3113 + t2713 * t4074 + (-0.1e1 * t2087 * t3801 + t2088 * t2630) * t3099 + ((-0.1e1 * t2977 * t2621 + t3905) * t3774 + t4116 * t2623) * t3103 + (t2630 * t4116 + t2943 * t3801) * t4361 + t4216 * t2087 * t4092 + t4211 * t4117 * t4093 + (t2803 * t3783 + t4066 * t4110) * t2620 - 0.50000000000000000000000000000000e0 * (t1527 * t2626 + t2064 * t3798 + t3034 + t3844) * t3778 + ((-0.1e1 * t2621 * t3520 - 0.1e1 * t2628 * t4220) * t4197 - 0.1e1 * t2943 * t3106 + (-0.1e1 * t2977 * t2621 + t2970) * t3107) * t2622 + 0.16143020000000000000000000000000e1 * (t4324 * t4322 - 0.1e1 * t1736 * t2630) * t4190 - 0.16143020000000000000000000000000e1 * (((-0.27518e-1 * t2630 + 0.39252e-1 * t3801) * t2628 + (0.39252e-1 * t2630 + 0.27518e-1 * t3801) * t2621) * t2630 + t2623 * (-0.1e1 * t2523 * t3774 + t3117 * t2623)) * t4281;
  t2907 = t1807 * t2612 + t1726 - t4086 - t4233;
  t1256 = t1906 + t2907 + t4152;
  t3305 = t3511 + t4043;
  t1296 = t2628 * t3305 - 0.21447119530300000000000000000000e-1 * t2621 + t3754;
  t1551 = t1720 + t4138;
  t1411 = t1551 * t2618 + t1972 * t2619 + 0.36044563611157510600000000000000e0;
  t1845 = t2025 * t2619 - 0.56786982094425000000000000000000e-2;
  t1583 = t1845 * t2628 - t1986 * t3818;
  t1886 = 0.32979938106866070000000000000000e-2 - t3747;
  t2324 = 0.3122837745659893e-2 * t2611 + 0.2333041922741103e-2;
  t3154 = -t1726 - 0.80863245317250000000000000000000e-1;
  t2760 = t2620 * t2890 + t3154 - t3957;
  t1445 = -0.27050000000000000000000000000000e-2 + t1639 - t3667;
  t3328 = t1445 * t2612 + t1468 - t3184 - t3966;
  t2924 = t3328 + 0.4741755542971769000000000000000e-2;
  t2926 = -0.1e1 * t1970 - t4140;
  t3242 = 0.56786982094425000000000000000000e-2 * t2619;
  t1875 = t3242 - t2025;
  t2979 = t1875 * t2618 + t4098;
  t3045 = t2509 - t1815;
  t3223 = 0.21751134959804000000000000000000e-1 * t2621;
  t3079 = t2619 * t3223;
  t3224 = 0.13297019103287584000000000000000e-1 * t2621;
  t3226 = 0.46305794820080000000000000000000e-2 * t2621;
  t3245 = 0.12089329343850000000000000000000e-2 * t2619;
  t2289 = t2621 * t3214;
  t1624 = t1986 * t2628 - t2236 * t2621 - t2289;
  t1327 = t1624 * t2625 + t3888 + (-0.23898270415101870000000000000000e-1 - t4317) * t2621 + t3755;
  t3165 = 0.56786982094425000000000000000000e-2 * t2628;
  t1427 = t2619 * t3380 - t3165;
  t3362 = t1327 * t2626 + t1427 * t2625;
  t1608 = -t1962 * t2628 - t2619 * t3668;
  t1258 = t1608 * t2625 + t2076 + (t2619 * t4235 + 0.55993270925625000000000000000000e-2) * t2621 + t3750;
  t2814 = -0.1e1 * t3985 - t2883;
  t1443 = t2621 * t2814 + t3584;
  t3363 = t1258 * t2626 + t1443 * t2625;
  t2680 = (-t2890 * t3842 + ((t1604 + t4051) * t2628 + (t2619 * t2926 + 0.1644487577369270e-2) * t2621 + t3362) * t2627 + (-t1605 * t2628 + (t2979 - 0.1e1 * t3245) * t2621 + t3363) * t2620 + t1296 * t2626 + t1583 * t2625 + t1411 * t2628 - 0.1e1 * t2618 * t3079 + t2619 * t3226 - 0.1e1 * t3224) * t4058 + t3045 * t3613 + t2760 * t3611 + (t1256 * t2613 + t1886 * t2605 + t2324 * t2612 + t2606 * t2924 + t3725 + 0.69005519272293457500000000000000e0) * t4065;
  t1005 = t2646 + t2680;
  t1455 = -t1990 * t3832 + t2762;
  t2181 = -0.68200000000000000000000000000000e-3 - t3263;
  t1570 = 0.42340000000000000000000000000000e-2 + t2181 * t2618 + t3764;
  t1267 = t1455 * t2612 + t1570 * t3826 + t2018 * t2611 + t3053;
  t3019 = t2334 + t3198;
  t1613 = t2618 * t3019 + t3994 - 0.8468e-2;
  t1269 = t1613 * t2612 + t4327;
  t1888 = -0.56440000000000000000000000000000e-2 - t2825;
  t1979 = -0.43600000000000000000000000000000e-3 + t2848;
  t1477 = t1979 * t2611 + t1888 * t3832 + 0.82920000000000000000000000000000e-2 + t3720;
  t1975 = -t3205 + t2181;
  t3031 = t1975 * t2625 + 0.45800000000000000000000000000000e-3;
  t1306 = -0.15592000000000000000000000000000e-1 + t1477 * t2626 + (-t3991 + t3031) * t2619;
  t3272 = 0.28220000000000000000000000000000e-2 * t2611;
  t1800 = -t3666 - t3272;
  t2855 = t3934 - 0.1e1 * t3669 + t2471 + t2335;
  t2771 = t2619 * t2855 + t4239 + 0.17282e-1;
  t2844 = t2875 * t2627;
  t1016 = t2523 * t2629 * t3491 + ((t2841 + (-t2521 * t2620 - t2844) * t2621) * t2629 + t3574) * t3496 - (-t2629 * t4102 + t2552) * t3492 + ((t4310 + (-t2620 * t2834 + t2627 * t2740) * t2621) * t2629 + t3574) * t3543 + ((-t2970 + (-t2627 * t3120 - t2571) * t2621) * t2629 + t3736) * t3494 + (t1306 * t3821 - t2908 + (t1267 - t1800) * t2613) * t3812 + t4134 * t4190 * t4301 + t4126 * (t2622 * t4102 - t3445) + (-t3396 - t3395) * (-t3445 + (t2621 * t4135 + t2970) * t2622) + (-t3399 - t3400) * (-t2621 * t2549 + t3445 + (t2841 + (-t2844 - t2226) * t2621) * t2622) + t4125 * (-t3445 + (t2621 * t2709 - t4310) * t2622) + (t4078 + t4073) * (-0.9522e-2 + t1269 * t2627 + t2771 * t2620);
  t3368 = -t1005 * t2637 + t1016 * t2636;
  t1610 = -0.1e1 * t3935 - t1827;
  t2856 = t3937 - 0.1e1 * t3670 + t3207 + t2336;
  t2774 = t1610 * t2626 + t2619 * t2856 + 0.8641e-2;
  t2798 = -t2618 * t3213 - t1599 + t3560 + t3660 + t3996;
  t2971 = t2628 * t3369;
  t3143 = -0.1e1 * t3871 + t3532;
  t3035 = t3143 * t2629;
  t3036 = t2621 * t3143;
  t3042 = t2628 * t3295;
  t3297 = t4278 * t2621;
  t3298 = t2628 * t4278;
  t3299 = t2621 * t3369;
  t3358 = t4008 - t4030;
  t2645 = (t2622 * t3042 + t4251) * t3107 + ((t3369 * t3778 + t4182) * t2623 + t2630 * t3299) * t3099 + ((t2622 * t3142 + t2629 * t3042) * t2630 + t2623 * t3036) * t3103 + ((-t2629 * t2971 - 0.1e1 * t4182) * t2630 + t2623 * t3299) * t3100 + t1337 * t3470 + (-0.1e1 * t2798 * t2620 + t2774 * t2627) * t4065 + ((-0.2e1 * t2749 * t3821 + t4118 * t1337) * t3809 - 0.1e1 * t2620 * t2755 - 0.1e1 * t3068 * t3787 + t3560 * t3779 + t4110 * t2627) * t4060 - 0.50000000000000000000000000000000e0 * (-0.1e1 * t2923 * t2620 + t2766 * t2627) * t3811 - 0.1e1 * (-0.1e1 * t4251 - 0.1e1 * t3295 * t3806) * t3106 + t2606 * t2818 * t4066 + t2803 * t3843 + ((t2622 * t4135 + t2628 * t3035) * t2623 + t2630 * t3036) * t4361 - 0.1e1 * ((t2622 * t3354 - 0.1e1 * t4278 * t3778) * t2630 + t2623 * t3297) * t3105 - 0.1e1 * ((t2629 * t3298 + (t2226 + 0.1e1 * t4312) * t2622) * t2623 + t2630 * t3297) * t3104 - 0.1e1 * (t3358 * t3777 + (t3358 * t3778 + (t4243 + t4029) * t2622) * t2623) * t3111 - 0.1e1 * ((0.1e1 * t4005 + t4242) * t3804 + ((-0.1e1 * t4242 - 0.1e1 * t4005) * t3778 + (-0.1e1 * t4243 + t4004) * t2622) * t2630) * t3113 + t4211 * (0.83327750000000000000000000000000e0 * t2629 * t3354 + t3298 * t4093) + t4216 * (0.17939475000000000000000000000000e1 * t2629 * t3119 - t2971 * t4092) + ((-0.1e1 * t1725 - t4352) * t2629 + (-0.1e1 * t4353 + t4008) * t3806) * t4197;
  t1391 = t1484 * t2620 - t3984;
  t1428 = t1531 * t2628 - t3889;
  t1444 = t1641 + t3667 - 0.23330419227411030000000000000000e-2;
  t1802 = -t2275 - t3876 - 0.23901105529490700000000000000000e-2;
  t1491 = t1802 * t2628 + t2621 * t2810;
  t1635 = t1744 * t2628 + t3223;
  t1510 = t1635 * t2627 + (0.52863517876992000000000000000000e-1 - t2460) * t2621;
  t1652 = t2621 * t2811 - 0.16444875773692700000000000000000e-2 * t2628;
  t1691 = t2165 * t2621 + t2076 + t2288;
  t1713 = -t2628 * t3044 - t3887;
  t1834 = t3382 + t3876;
  t2358 = -0.3344965323567556e-2 * t2617 - 0.187138194629210e-3;
  t2866 = (t2358 - t3383) * t2619 + 0.11357396418885000000000000000000e-1;
  t2930 = t2620 * t3525 + t2627 * t3522;
  t2077 = t2172 * t2620;
  t2978 = t1388 * t2625 - t2627 * t3511 - t2077;
  t3004 = -t2480 - 0.1e1 * t2179;
  t2676 = 0.82224378868463500000000000000000e-3 * t3807 + (t3514 * t4257 + (t1428 * t2620 + t3524 * t2625 + (t3785 * t4235 + t1713) * t2627) * t2626 + t1444 * t3852 + (t1391 * t3792 + t1691 * t2627 + t2620 * t3381) * t2619 + t1510 * t2625 + t1491 * t2627 + t1652 * t2620 - 0.1e1 * t2177 * t3819 + ((t2618 * t2866 + t2925) * t2626 + t3004 * t2619 + t2184 + t4302) * t2621) * t4058 + t2930 * t3612 + t2978 * t3621 - t3606 * t4316 + (t1834 + t4040) * t3613;
  t1007 = t2645 + t2676;
  t2843 = t2875 * t2629;
  t1018 = t2620 * t1990 * t3662 + ((t2521 * t3778 + t2845) * t2627 + (t2521 * t2622 - t2628 * t2843) * t2620 + t3455) * t3496 + (-0.1e1 * t1269 * t2620 + t2771 * t2627) * t3615 + (t1267 * t3708 + t1306 * t4118) * t4077 - ((t2628 * t3530 + t3564) * t2627 + (-0.1e1 * t2628 * t3562 + t3539) * t2620) * t3492 + ((-t2622 * t2740 + t2834 * t3778) * t2627 + (t2622 * t2834 + t2740 * t3778) * t2620 + t3455) * t3543 + ((t2622 * t3120 + t2628 * t3529) * t2627 + (-0.1e1 * t3120 * t3778 + t3537) * t2620 + t3735) * t3494 + (-0.1e1 * t1800 * t2614 - 0.1e1 * t3272) * t3821 + t4126 * ((-t2628 * t3539 + t3562) * t2627 + (t2628 * t3564 + t3530) * t2620) + t4114 * ((t2356 * t2629 - t3413) * t2627 + (t2356 * t3806 + t3529) * t2620) + t4113 * (-t2622 * t3446 - t3444 + (t2354 * t3806 - t2843) * t2627 + (-t2354 * t2629 - t2628 * t2845) * t2620) + t4125 * ((t2629 * t2734 - t3806 * t4105) * t2627 + (t2629 * t4105 + t2734 * t3806) * t2620);
  t3367 = -t1007 * t2637 + t1018 * t2636;
  t1338 = -0.1e1 * t1528 * t2619 + t4239;
  t1649 = -t3760 - t4256;
  t2129 = 0.41065000000000000000000000000000e-1 * t2619 + 0.11953000000000000000000000000000e-1 * t2626;
  t3313 = t2129 * t2628 - t2522 * t3813;
  t3314 = t2628 * t2875 + t3300 * t3813;
  t2649 = (t3680 - t4293) * t3106 + (((t2005 - t3940) * t2629 + t4172) * t2623 + t3314 * t2630) * t3104 + (((-0.1e1 * t2005 + t3940) * t2629 - 0.1e1 * t4172) * t2630 + t3314 * t2623) * t3105 + ((t1649 * t2628 - t3329 * t3813) * t2623 + ((t1649 * t2621 + t3329 * t3783) * t2629 + t3329 * t3810) * t2630) * t3113 - ((-t4104 * t2629 - 0.1e1 * t3679) * t2623 + t3313 * t2630) * t3102 + ((-t3704 + (t2537 - 0.1e1 * t4122) * t2621) * t3801 + (-0.1e1 * t2537 + t4122) * t3775 - (t2627 * t3777 + t3653) * t4220) * t3111 + ((-0.1e1 * t3854 + t1462 + 0.2e1 * t1581) * t2627 + (-0.1e1 * t1610 * t2619 + t2856 * t2626) * t2620) * t4064 + ((t1268 * t2613 + t1338 * t3821 + t1268) * t3809 + (-0.1e1 * t1609 * t2619 + t2840 * t2626) * t3779 + 0.2e1 * t1618 * t3472 + t1480 * t3672 - 0.1e1 * t3782 * t3854) * t4059 + ((t1614 * t3706 - t4336) * t2627 + (-0.1e1 * t1611 * t2619 + t2839 * t2626) * t2620) * t3614 - 0.1e1 * (t4293 - 0.1e1 * t3680) * t3107 + t1338 * t3462 + t1527 * t3458 - 0.1e1 * (((t2129 * t2621 + t2204) * t2629 + t3679) * t2630 + t3313 * t2623) * t3103 + (-0.2e1 * t3660 + t3711 * t1618) * t3371 + t1609 * t3457 + t4225 * (t2005 * t2622 - t2621 * t2845 - t4244) + t4224 * (t4220 * t3782 + (t2621 * t4156 - t3704) * t2622);
  t3169 = 0.21751134959804000000000000000000e-1 * t2627;
  t2847 = -t3169 + t2460;
  t2782 = t2847 - 0.26431758938496000000000000000000e-1;
  t2765 = t2782 * t2621;
  t1495 = -t1744 * t3783 + t2765;
  t2886 = -0.1e1 * t1909 - t3970 + t3050;
  t2717 = t2621 * t2769 + t2628 * t2886 - t2294;
  t2783 = -t3168 + t3146;
  t2889 = t4275 * t2621;
  t1509 = -t2628 * t2783 + t2889;
  t2733 = t1509 * t2618 + t2823 * t2628 - t2293 + (0.1e1 * t3981 - t3970 + t2158) * t2621;
  t3144 = t2513 - 0.12089329343850000000000000000000e-2;
  t2905 = t3144 + t3967 - t3974;
  t3310 = t3640 - t3818;
  t2916 = -t1968 * t3310 + t1971 * t3784;
  t2917 = t3044 + t3506;
  t1316 = -t2289 - t2084 + ((t4024 - 0.1e1 * t1978) * t2627 - t4158) * t2628;
  t3007 = -0.1e1 * t2161 - t2469;
  t2859 = -0.1e1 * t1932 - 0.1e1 * t1903 + t3007;
  t1374 = -0.1e1 * t2003 * t3783 + t2859 * t2621;
  t1469 = t1694 * t3818 + t1968 * t3784;
  t3125 = t1316 * t2626 + t1374 * t2619 + t1469 * t2618;
  t3315 = t1971 * t2627 + t3692;
  t3132 = t3315 * t2611;
  t1686 = t3984 + t4138;
  t1357 = t2620 * t4166 + t1686;
  t3138 = t1357 * t2626 + t2003 * t3823 + t1871;
  t3164 = 0.23126197987767817000000000000000e-1 * t2628;
  t2674 = (t1495 * t3835 + t2604 * t3698 + t2611 * t2916 + t2619 * t2717 + t2620 * t3164 + t2625 * t3125 + t2626 * t2733) * t4058 - 0.11563098993883908500000000000000e-1 * t3807 + t3132 * t4065 + t3138 * t3606 + t2905 * t3612 + t2917 * t3621 + t3611 * t3988 + t3463 * t3828;
  t1009 = t2649 - t2674;
  t2723 = (t2524 * t2621 + 0.10517e-1 * t3783) * t2626 + (t2524 * t3783 - 0.10517e-1 * t2621) * t2619;
  t2737 = t2620 * t2741;
  t2972 = t2522 * t2620;
  t2974 = t2627 * t3123;
  t1024 = (t2629 * t2723 + t4172) * t3496 + ((t1613 * t3706 + t4336) * t2627 + (-0.1e1 * t4240 + t2855 * t2626) * t2620) * t3615 + (-0.1e1 * t1477 * t2619 * t3821 + t3711 * t2613 * t1570 + (t1455 * t2613 * t4082 + (t2618 * t4213 + t3031 + t3255) * t3821) * t2626) * t4077 + t1268 * t4073 + (t2622 * t2737 + ((t4255 - 0.1e1 * t3123 * t3783) * t2626 + t4288) * t2629) * t3543 + (-t2622 * t2972 + (-0.1e1 * t4186 + t4179) * t2629) * t3494 + t4114 * (-t2629 * t2972 + (-t4179 + t4186) * t2622) + t4113 * (t2622 * t2723 - t4244) + t4125 * (t2629 * t2737 + ((t2628 * t2974 - t4255) * t2626 - t4288) * t2622);
  t3366 = t1009 * t2637 + t1024 * t2636;
  t2745 = -0.1e1 * t3939 + t3990;
  t1328 = (0.2e1 * t1948 - 0.1e1 * t2604 * t1897 + t1854) * t2626 + t2745 * t2619;
  t1756 = t2951 * t2619;
  t1757 = t2951 * t2626;
  t1787 = t1966 * t2625 + t3248;
  t3284 = -0.1e1 * t3869 + t3552;
  t1957 = t3284 * t2626;
  t2858 = 0.2e1 * t2065 * t3475 + (t3675 - t3676) * t1897;
  t2941 = -0.1e1 * t3979 + t3183;
  t2942 = t2521 * t3818;
  t3294 = -t4108 + t3771;
  t2648 = (((t1852 - 0.1e1 * t3903) * t2629 + t4171) * t2623 + (t2152 * t2628 + t2621 * t3312) * t2630) * t3104 + (((t3903 - 0.1e1 * t1852) * t2629 - 0.1e1 * t4171) * t2630 + t2152 * t3802 + t2521 * t2623 * t3648 + t2524 * t3645) * t3105 + ((t2619 * t3284 * t3804 + t1757 * t3644 + t1787 * t3651) * t2629 + (t1757 * t3777 - 0.1e1 * t3301 * t3803) * t2627 + t2834 * t2619 * t3775 + t1757 * t3653 + t1787 * t3633) * t3111 + ((t1756 * t2621 + (t1957 * t2627 - 0.1e1 * t3301 * t2620) * t2628) * t3774 + (t2626 * t2834 * t3804 + t3301 * t3776) * t2627 + t1957 * t3652 + t1756 * t3802 + t3301 * t3645) * t3113 + ((t1623 * t2612 + t1512 * t3826 - 0.1e1 * t3997 + (t2339 - 0.1e1 * t3213) * t2625) * t2627 + (t3936 + t3996) * t3791 + t2063 * t3411 + (-0.1e1 * t3675 + t3676) * t1884) * t4064 + (((t3407 + t3771) * t2613 + t1328 * t3821 + t3294) * t3809 + ((-0.1e1 * t3936 - 0.1e1 * t3996) * t2626 + 0.2e1 * t2063 * t3663 + t1884 * t3850 - 0.1e1 * t2619 * t3993) * t3779 + t1623 * t3672 + t1512 * t3472 - 0.1e1 * t1882 * t3661 - 0.1e1 * t2625 * t2994 + t2339 * t3641) * t4059 + (((t2625 * t3002 + t3995) * t2612 - t4309) * t2627 + (t3939 - 0.1e1 * t3990) * t3791 + t2858) * t3614 + t1328 * t3462 + (-0.1e1 * t3992 - 0.2e1 * t3666 + t3993) * t3457 + t2064 * t3373 + (t1512 * t2612 + t1512 - t4321) * t3371 + t3458 * t3996 + t4225 * ((t1852 - t2942) * t2622 - t3311 * t2629) + t4224 * ((t1787 * t2627 + t2941 * t3791) * t2629 + t2941 * t3646 + (t1757 * t3783 + t1787 * t3784) * t2622);
  t2752 = -t3984 + t1962 - t3968;
  t2867 = -t2201 - 0.5483591064082320000000000000000e-3 * t2624;
  t2837 = t2626 * t2867;
  t2712 = t2619 * t2752 + t2620 * t2837 + t4013;
  t3176 = 0.26431758938496000000000000000000e-1 * t2626;
  t2780 = t3176 + 0.13609823097337500000000000000000e-1 + t2478;
  t3177 = 0.56786982094425000000000000000000e-2 * t2626;
  t2880 = -0.52129746651620000000000000000000e-1 - t3177;
  t2863 = -t3268 + t2880;
  t2830 = t2863 * t2620;
  t2719 = t2423 + t2830 + t2780;
  t2313 = t2620 * t3165;
  t3163 = 0.26431758938496000000000000000000e-1 * t2628;
  t2894 = t2627 * t3163 - t2313 + t3584;
  t2953 = -t3043 + t4232;
  t2920 = t2953 * t2627;
  t2732 = (-t2621 * t2883 + t2894) * t2625 - t2628 * t2920;
  t2772 = t3897 - t4221;
  t2759 = t2626 * t2772;
  t2743 = t2003 * t2627 + t2620 * t2759;
  t2802 = t4097 * t2627;
  t2862 = t2512 - t4089;
  t2829 = t2862 * t2627;
  t2981 = t3731 + t4200;
  t2954 = -t3892 + t2981;
  t2922 = t2954 * t2620;
  t2861 = t1983 * t2625 + t2922;
  t2870 = t2621 * t4198 + t3509;
  t3356 = -t1918 + t1903;
  t2915 = -t2628 * t3356 + t3403;
  t3027 = -t2161 * t2626 + 0.56786982094425000000000000000000e-2;
  t3069 = t2626 * t2469;
  t3285 = 0.5483591064082320000000000000000e-3 * t2628;
  t2130 = -t3227 + t3285;
  t3349 = t2130 * t2624 + t3879;
  t3124 = t3349 + t3882;
  t3225 = 0.56786982094425000000000000000000e-2 * t2621;
  t2519 = 0.54835910640823200000000000000000e-3 * t2628;
  t2127 = -t3227 + t2519;
  t3350 = t2127 * t2624 + t3879;
  t3296 = t3350 * t2620;
  t2652 = t2861 * t3621 + t2743 * t3606 - t2712 * t3833 / 0.2e1 + ((t2915 * t2619 + (t2626 * t3124 - t3225) * t2627 + (t2870 - t3883) * t2620) * t2618 + t2732 * t2619 + (t2802 + t3296) * t2625 + ((-t3069 + t3027) * t2618 + (t2829 + t2719) * t2625 + t4208) * t2621) * t4058;
  t1012 = t2648 - t2652;
  t2929 = t2359 * t2627;
  t2720 = (-t2620 * t3548 - t2929) * t2625 + (t2626 * t2928 - t3545) * t2618;
  t2721 = -t2942 + ((-t2626 * t3547 + t3555) * t2625 + (t2626 * t3546 + t3556) * t2618) * t2628;
  t1026 = t3274 * t3832 + t3092 * t3832 + t3954 * t4079 + (t2622 * t4096 + t2629 * t2721) * t3496 + (((-0.1e1 * t3995 + t3019 * t2625) * t2612 + t4309) * t2627 + t2745 * t3791 - 0.1e1 * t2858) * t3615 + (((t3955 - 0.1e1 * t3954 + t1803) * t2612 + t2018 * t3707) * t2613 + (t1979 * t3707 + (-0.1e1 * t2604 + t2611) * t1888) * t3650 + ((-0.1e1 * t3991 + t2181 * t2625 - 0.1e1 * t2306) * t2626 * t2613 + (-0.1e1 * t1975 * t2618 + (0.14600000000000000000000000000000e-2 + t4213) * t2625) * t3821) * t2619) * t4077 + ((t3503 + 0.56440000000000000000000000000000e-2 * t3832) * t2613 + t3294) * t4073 + (t2720 * t2622 + (-0.1e1 * t4249 + ((t2928 - 0.1e1 * t3440) * t2625 + (t2359 * t3790 + t3554) * t2618) * t2628) * t2629) * t3543 + (-0.50000000000000000000000000000000e0 * t3955 + 0.28220000000000000000000000000000e-2 * t3832) * t2606 + t4113 * (t2622 * t2721 - t2629 * t4096) + t4125 * (t2720 * t2629 + (t4249 + ((t3440 - t2928) * t2625 + (-t2626 * t2929 - t3554) * t2618) * t2628) * t2622);
  t3365 = t1012 * t2637 + t1026 * t2636;
  t2738 = 0.1e1 * t3921 + t4195;
  t1339 = (-0.1e1 * t3925 - 0.1e1 * t3671 + t2106) * t2626 + t2738 * t2619;
  t1731 = t2098 * t3793 - t2128 * t2619;
  t1784 = t2320 + t3659;
  t1900 = -t3123 * t3793 + t3860;
  t2735 = t2620 * (-t3921 - t4195);
  t2736 = t1855 * t3475 + t2101 * t3675 - t2106 * t3823;
  t2750 = t1857 + t3773;
  t2779 = t2626 * (-t2618 * t3720 + t1824);
  t2792 = t1855 - t3999 - t4295;
  t3075 = t2620 * t3213;
  t3093 = t2619 * t3267;
  t3133 = (t1731 * t2627 - t2098 * t3834) * t2628;
  t3316 = t2101 * t3832 - t4000;
  t2647 = ((t1784 * t2621 + (t1900 * t2627 + t4173) * t2628) * t3774 + (-0.1e1 * t1900 * t3804 - 0.1e1 * t2630 * t3678) * t2627 + t1900 * t3652 + t1784 * t3802 - 0.1e1 * t3123 * t2618 * t3645) * t3113 + ((t2621 * t4123 + t3133) * t3801 + (t1731 * t3777 + t2623 * t3678) * t2627 - 0.1e1 * t4123 * t3775 + t1731 * t3653 - 0.1e1 * t2098 * t2618 * t3633) * t3111 + ((t1622 * t2612 + t1860 * t2625 + t2115 * t2618 - t3826 * t4160) * t2627 + (-0.1e1 * t3917 + t4194) * t3791 + t1857 * t3475 - 0.1e1 * t2619 * t3075 + (t3658 - 0.1e1 * t3093) * t2620) * t4064 + (((-t1855 + t3765 + t3773) * t2613 + t1339 * t3821 + t2750 + t3316) * t3809 + ((t3917 - 0.1e1 * t4194) * t2626 - 0.1e1 * t3658 - 0.1e1 * t1857 * t3663 + t3093 + t2619 * t3213) * t3779 + t1622 * t3672 - t4160 * t3472 + t1860 * t3641 + t2115 * t3661) * t4059 + (((t4180 + t4187) * t2612 + (t1855 - 0.1e1 * t3316) * t3826 + t1622) * t2627 + t2626 * t2735 - 0.1e1 * t2736) * t3614 + t1339 * t3462 + (t1857 * t3832 + t2106 * t2611 + t2851) * t3457 + t2115 * t3591 * t3818 + (t2619 * t2779 + t2792 + t3664) * t3371 + t1860 * t3373 + t4224 * ((-t1731 * t2620 - t2098 * t3787) * t2629 + ((-t2128 * t2626 - t3659) * t2621 + t3133) * t2622);
  t2763 = -t4103 - 0.6381775021050e-3;
  t3172 = 0.16724826617837780000000000000000e-2 * t2627;
  t3062 = t2618 * t3172;
  t3239 = 0.54835910640823200000000000000000e-3 * t2620;
  t2807 = t2619 * t3239 + t3062;
  t2944 = t3378 - 0.735522e0 * t3388;
  t2707 = t2625 * t2944 + t2626 * t2763 - t2807;
  t3191 = 0.54835910640823200000000000000000e-3 * t2625;
  t2902 = t3191 + t3454;
  t2764 = t2620 * t2902 + t3428 - 0.2580137623800e-3;
  t3173 = 0.54835910640823200000000000000000e-3 * t2627;
  t3063 = t2618 * t3173;
  t3237 = 0.16724826617837780000000000000000e-2 * t2620;
  t2806 = t2619 * t3237 - t3063;
  t2945 = t3379 + 0.735522e0 * t3387;
  t2708 = t2625 * t2945 + t2626 * t2764 - t2806;
  t2876 = -t2949 - 0.2970426191616e-2;
  t2754 = t2621 * t2876 - t2627 * t3285;
  t3228 = 0.16724826617837780000000000000000e-2 * t2621;
  t2897 = -0.988270895904e-3 * t2628 + t3228;
  t3340 = t2628 * t3454;
  t2710 = t2620 * t3424 + t2625 * t2754 - t2627 * t3340 + t2897;
  t3015 = 0.1200936784896e-2 - t3435;
  t2877 = -0.1e1 * t3878 + t3015 * t2621;
  t3339 = t2628 * t3453;
  t2731 = t2620 * t3423 + t2625 * t2877 - t2627 * t3339 + t3713;
  t2748 = -t3283 * t3414 + (t2628 * t3016 - t3228) * t2619;
  t2896 = t2519 + t3431;
  t2786 = t2618 * t2896 - t2619 * t3433;
  t2787 = t2205 * t2618 - t2619 * t3432;
  t2816 = t2557 * t3414 + (-t2628 * t3425 + t3713) * t2619;
  t3336 = t2618 * t3433;
  t2868 = t2619 * t2896 - t3336;
  t3335 = t2618 * t3432;
  t3013 = -t2205 * t2619 + t3335;
  t3189 = 0.49096519673609460000000000000000e-2 * t2625;
  t3066 = t2620 * t3189;
  t3222 = 0.24548259836804730000000000000000e-2 * t2622;
  t3343 = t2621 * t3453;
  t3344 = t2621 * t3454;
  t2650 = t3222 * t3786 + ((t2619 * t3343 + t2620 * t2787 + t2625 * t2748 + t2626 * t2731 + t2627 * t2868 + t3336) * t2624 + (t2619 * t3344 + t2620 * t2786 + t2625 * t2816 + t2626 * t2710 + t2627 * t3013 - t3335) * t2617 - t2628 * t3066) * t4058 + (t2617 * t2708 + t2624 * t2707) * t4065 + (-t3222 * t3791 + t4058 * t4131) * t2618;
  t1014 = t2647 - t2650;
  t2722 = t2618 * t2974 + t2620 * t2776;
  t1035 = t2604 * t3090 + t2606 * t2106 * t3625 - 0.50000000000000000000000000000000e0 * (((-0.1e1 * t4187 - 0.1e1 * t4180) * t2612 + (t3316 - t1855) * t3826 - 0.1e1 * t2271 - t4161) * t2627 + t2738 * t3791 + t2736) * t3812 + (t2792 * t2613 + (t3671 + t3925 - t2106) * t3650 + (t2613 * t2779 + t2627 * t2735) * t2619) * t4078 + (-0.1e1 * t4000 + (-0.1e1 * t2106 * t2613 + t2101) * t3832 + t2750) * t4074 - 0.1e1 * (t2722 * t2622 + ((-0.1e1 * t4188 + t4181) * t2621 + (t4178 - 0.1e1 * t4173) * t2628) * t2629) * t3543 + 0.42800000000000000000000000000000e-3 * (-0.1e1 * t2610 + t2603) * t2604 + (-0.1e1 * t2609 - 0.1e1 * t2616) * (t2722 * t2629 + ((-t4181 + t4188) * t2621 + (t4173 - t4178) * t2628) * t2622) * t3542;
  t3364 = t1014 * t2637 - t1035 * t2636;
  t2026 = t2479 + 0.26595745882176000000000000000000e-4 * t3838;
  t3326 = -t4209 + t4264;
  t3361 = (t2026 * t2618 + t3326) * t2625 + t2027;
  t1545 = t3948 + t4347;
  t2124 = t3170 + t3232;
  t3355 = -t2124 * t2618 - t3974;
  t3351 = t2619 * t3724 + t2812;
  t2176 = 0.31600000000000000000000000000000e0 - t3231;
  t3345 = t2176 * t3452;
  t3342 = t2627 * t3454;
  t3341 = t2627 * t3453;
  t3338 = t2618 * t3424;
  t3337 = t2618 * t3423;
  t3334 = t2620 * t3433;
  t3333 = t2620 * t3432;
  t3332 = t2621 * t3430;
  t3331 = t2621 * t3429;
  t3327 = -t4320 - t4284;
  t3320 = t2618 * t3383;
  t1370 = t1639 + t2955;
  t3308 = t1370 * t2612 + t1853 + t3370 + t4090;
  t3005 = t2386 - 0.1e1 * t2017;
  t1499 = t2618 * t3005 - t4283;
  t3306 = t1499 * t2625 + t3511;
  t3303 = -0.3030488946654060e-2 + t3900;
  t1806 = 0.2e1 * t3700;
  t3293 = t2612 * t3083 + t1771 + t1806 + t3508;
  t3287 = 0.5483591064082320000000000000000e-3 * t2621;
  t3286 = 0.5483591064082320000000000000000e-3 * t2625;
  t3282 = 0.50000000000000000000000000000000e0 * t1707;
  t3280 = 0.50000000000000000000000000000000e0 * t2852;
  t3276 = 0.39510871831575200000000000000000e-3 * t2610;
  t3256 = 0.54835910640823200000000000000000e-3 * t2618;
  t3254 = 0.49096519673609460000000000000000e-2 * t2618;
  t3247 = 0.51602752476000000000000000000000e-3 * t2619;
  t3246 = 0.54835910640823200000000000000000e-3 * t2619;
  t3244 = 0.16724826617837780000000000000000e-2 * t2619;
  t3240 = 0.27417955320411600000000000000000e-3 * t2620;
  t3233 = 0.21751134959804000000000000000000e-1 * t2620;
  t3229 = 0.98827089590400000000000000000000e-3 * t2621;
  t3219 = 0.73552200000000000000000000000000e0 * t2623;
  t3217 = 0.32286040000000000000000000000000e1 * t2623;
  t3212 = 0.83624133089188900000000000000000e-3 * t2624;
  t3200 = 0.24209437785212300000000000000000e-2 * t2624;
  t3188 = 0.56786982094425000000000000000000e-2 * t2625;
  t3187 = 0.21751134959804000000000000000000e-1 * t2625;
  t3186 = 0.26431758938496000000000000000000e-1 * t2625;
  t3182 = 0.28244044800000000000000000000000e0 * t2625;
  t3180 = 0.25801376238000000000000000000000e-3 * t2626;
  t3179 = 0.54835910640823200000000000000000e-3 * t2626;
  t3178 = 0.16724826617837780000000000000000e-2 * t2626;
  t3174 = 0.25801376238000000000000000000000e-3 * t2627;
  t3171 = 0.49096519673609460000000000000000e-2 * t2627;
  t3162 = 0.24548259836804730000000000000000e-2 * t2629;
  t3159 = 0.73552200000000000000000000000000e0 * t2630;
  t3157 = 0.32286040000000000000000000000000e1 * t2630;
  t3156 = 0.3122837745659893e-2 * t2612 * t3832;
  t3145 = -t3233 + 0.56786982094425000000000000000000e-2;
  t3141 = t1821 + t1822 + t3686 + t3456;
  t3140 = 0.3507900e-3 * t4298;
  t3139 = 0.8676525e-3 * t4298;
  t3137 = -t4235 + t3667;
  t3134 = t1697 * t2611 + t3667 - 0.2333041922741103e-2;
  t2315 = t2628 * t3216;
  t2655 = ((0.1e1 * t4346 - 0.1e1 * t1832) * t3813 * t2612 + ((t2358 * t3830 + t3668 * t3786 + t3813 * t4115) * t2619 + (0.1e1 * t3044 * t2621 - 0.1e1 * t2076) * t2627 + ((-0.1e1 * t2025 * t2621 + t2083) * t2625 - 0.1e1 * t1531 * t2621 - 0.1e1 * t3888) * t2620) * t2626 + (-0.1e1 * t1391 * t3796 + (t2315 - 0.1e1 * t3887) * t2627 + (t1833 * t2621 + t3691) * t2620) * t2619 + ((-0.1e1 * t4315 + t2517) * t2627 - 0.1e1 * t2313) * t2625 - 0.1e1 * t1802 * t3813 + 0.16444875773692700000000000000000e-2 * t3817 - 0.1e1 * t2177 * t3830 + (((t2931 * t2625 - 0.1e1 * t3320 + 0.3030488946654060e-2) * t2619 + ((-0.24444132201840000000000000000000e-2 * t2620 + 0.12763550042100000000000000000000e-2) * t2624 + t3504) * t2625 + t2171) * t2626 + t1444 * t2605 + (t3024 * t2620 - 0.1e1 * t1989 + t4192) * t2619 + t3184 + t4269 + t4302) * t2628) * t4064;
  t2939 = -t3045 * t2627 / 0.2e1;
  t2687 = (-0.1e1 * t3362 * t2620 + t3363 * t2627 + (t1155 * t2613 - 0.1e1 * t4266 + (0.2e1 * t2890 * t2627 - 0.1e1 * t1604 - 0.1e1 * t4051) * t2620) * t2628 + (-0.1e1 * t3384 + t2979 * t2627 + (-0.1e1 * t2926 * t2620 - 0.1e1 * t2513) * t2619) * t2621) * t4065 + t2629 * t2939 + t2760 * t3593 - 0.50000000000000000000000000000000e0 * t2890 * t3841 + (t1256 - 0.1e1 * t2924) * t3634;
  t1023 = t2655 + t2687;
  t2887 = t2627 * t4111;
  t2746 = t2620 * t3306 + t2626 * t2887 + t3507;
  t2770 = t3984 - t3047;
  t2753 = t2770 - t3964;
  t2813 = -0.1e1 * t1960 - t1531;
  t2777 = 0.1e1 * t1914 + t2813 * t2620;
  t2781 = -t2847 + 0.52863517876992000000000000000000e-1;
  t2865 = -t2078 + t2171;
  t2869 = t1519 * t2626 + t3049 + t4159;
  t3052 = -0.60029938106866070000000000000000e-2 + t3747;
  t2664 = (t1834 * t2627 + t2619 * t2746 + t2626 * t2777 + t4109) * t4059 + (t3134 * t2605 + t2869 * t2619 + t3052 * t2612 + (t2625 * t2753 + t2865 - t3890) * t2626 + t2781 * t2625 - t3347 - t2177 * t2618 + t4269) * t4067;
  t1716 = -t2619 * t3304 + t2171;
  t1734 = -t1809 * t2620 + 0.56786982094425000000000000000000e-2;
  t1432 = -t1556 * t2620 + t3022;
  t2965 = t1432 * t2625 - t2170;
  t1144 = t2965 * t2626 + t1734 * t2625 + (t1716 * t2626 + t3308) * t2620 - t1604;
  t1209 = t1538 + t3153 + t4169;
  t1870 = t1968 * t3850;
  t3054 = -t4317 + t2158;
  t2989 = -t2474 + t3054;
  t2956 = -t1960 + t2989;
  t1245 = t2956 * t2626 + t1870 + 0.1644487577369270e-2 + (t1833 + t4043) * t2619;
  t1543 = t1728 * t2619 - t3044;
  t1717 = t2172 * t2619 - t3947 - 0.2390110552949070e-2;
  t1797 = t2627 * t3476;
  t2700 = (t1209 * t3708 + ((t1716 - t4368) * t2626 - t4265 + t3308) * t2613 - t1144 * t2620 + (t1962 * t3786 - t2078) * t2626 - t2625 * t3169 + t4266) * t4066 + t1245 * t3597 + (-t1797 + (t1666 * t3850 + t1543) * t2627) * t3601 + (t1717 + t4039 + t4348) * t3595;
  t1031 = -t2664 + t2700;
  t2123 = t3247 + t3265;
  t1938 = t2156 * t2619 + 0.12763550042100000000000000000000e-2;
  t2824 = t1938 * t2624 + t2163;
  t3028 = t2157 + t3209;
  t2702 = -t4374 - t2509 + t2824 * t2618 + 0.27752814537092170000000000000000e0 + (t2618 * t3020 + t2625 * t3028 + t4300) * t2619;
  t1075 = -0.50000000000000000000000000000000e0 * t2702 * t2613 + (-0.1e1 * t2480 * t2619 + t2620 * t2702 + t3154 - 0.1e1 * t3884) * t4068 + t2939 + (t2123 * t2624 + t3950 + t2907 + t3884 - 0.4741755542971769e-2 - 0.1e1 * t3328) * t3821;
  t2635 = q_state_dot(3);
  t3129 = -t1023 * t2637 + t1031 * t2636 - t1075 * t2635;
  t3003 = -t3214 - 0.1e1 * t2201;
  t3055 = t2628 * t2474;
  t2662 = ((-t1971 * t3817 + (t3648 + t3785) * t1968) * t2611 + (((-0.1e1 * t1903 - t1986) * t2626 - 0.1e1 * t3693 + ((-0.1e1 * t4024 + t1978) * t2626 + t3952) * t2627) * t2621 + (t3003 * t2626 + (t2859 + t1660) * t2619) * t2628) * t2625 + ((t2621 * t2783 + t2628 * t4275) * t2618 - t2823 * t2621 + t3050 * t3783 - t3044 * t3784 - t3055 + t4193) * t2626 - t2621 * t3699 + (t2628 * t2782 + t3813 * t4299) * t3835 + (-0.1e1 * t2886 * t2621 + t4226 * t2628) * t2619 - 0.23126197987767817000000000000000e-1 * t3817) * t2622;
  t1233 = t1445 * t3709 + t1490 - t3853;
  t1701 = t1744 * t3831;
  t2857 = -0.1e1 * t3667 + t4235;
  t2672 = ((-0.1e1 * t4047 + (-0.1e1 * t1545 - 0.1e1 * t4300) * t2626) * t3842 + ((t1371 * t3709 + (t2626 * t3304 - t1702) * t2626 - 0.1e1 * t1373 * t2619 + t3758) * t3784 - 0.1e1 * t1327 * t2619 + t2626 * t3691 + t3380 * t3793 + t3050 * t4340 - 0.1e1 * t3176 * t3819 - 0.1e1 * t1970 * t3815) * t2627 + (t1529 * t2621 * t3709 - 0.1e1 * t1258 * t2619 - 0.1e1 * t1962 * t3642 + t3044 * t4340 + t2857 * t3814 + t3177 * t3819 - 0.12089329343850000000000000000000e-2 * t3815) * t2620 - 0.1e1 * t1296 * t2619 + (t3946 - 0.1e1 * t3963) * t3793 + (t1972 * t2626 + t1701) * t2628 - 0.1e1 * t2512 * t3819 + t2626 * t3226) * t4064 + t1233 * t3630 + (-0.1e1 * t3956 + (0.1e1 * t1348 * t2620 + 0.1e1 * t1755) * t2619 + t4168 * t3791) * t3590 + t4279 * t3627 + (t1886 - 0.1e1 * t2324) * t3656;
  t1027 = -t2662 / 0.2e1 + t2672;
  t2990 = t1667 * t2618 - t1978;
  t1416 = t1903 + t2990;
  t2761 = t1970 + t4140;
  t2747 = t1416 * t2625 - t2077 + t2761;
  t2794 = (t1543 + (t1639 - 0.1e1 * t3667) * t2619) * t2620 + t3050;
  t2673 = t1529 * t3473 + ((t2626 * t4168 + t4047) * t2613 + (t1370 * t3526 + (-0.1e1 * t3949 + t4099) * t4189 - (t1716 * t2620 + t2965) * t2619 - t3758 * t2620 - t3050 * t2626) * t2627 - t2747 * t2619 - t2025 * t3793 - t3044 * t3791 + t2989 * t2626) * t4067 + t2170 * t3601 - (-0.1e1 * t2956 * t2619 + t3305 * t2626) * t3783 / 0.2e1 + t2794 * t3598 + t3597 * t3886 + t2628 * t4158 * t3605 + t3137 * t3465;
  t2913 = t2176 * t3449 + 0.52129746651620000000000000000000e-1;
  t1353 = t2079 - t3268 - t2913 + t3770;
  t1281 = t1353 * t2626 + t3409;
  t1356 = t1660 - t1932 - t2019 + t2079 - t2161;
  t1936 = t2003 * t2626;
  t1321 = t1356 * t2619 - t1936;
  t1361 = t2176 * t3450 + t1909 - t2881 - t3891 + t4313;
  t1363 = -t2175 * t3450 + t3054 + t3891 + t3981;
  t1562 = t2618 * t2783 - t2823;
  t1984 = -t3169 - t4087;
  t1574 = t1984 * t2618 + t4226;
  t2718 = (t1281 * t2625 + t1361 * t2619 + t1562 * t2626 + t1603 * t2611 + t2620 * t4088) * t4059 + (t1363 * t2626 + t1574 * t2619) * t4067 - t1321 * t3796 / 0.2e1 + t3616 * t3851;
  t1039 = t2673 + t2718;
  t3095 = t2626 * t2385;
  t1098 = t4279 * t4075 + ((0.1e1 * t4047 + t3028 * t3793 + t1748 * t3831) * t2620 + t4339 + (t4300 * t2620 - 0.1e1 * t1989) * t2626) * t4061 + t1233 * t4079 - 0.1e1 * t2619 * t3095 + (-0.1e1 * t2324 - 0.1e1 * t2250 + 0.32979938106866070000000000000000e-2) * t3826;
  t3128 = t1027 * t2637 - t1039 * t2636 + t1098 * t2635;
  t2900 = t2627 * (-t3292 + t3500);
  t2658 = ((((-0.1e1 * t2182 + t3356) * t2621 - 0.1e1 * t3350) * t2619 + (-0.1e1 * t3165 + ((-0.1e1 * t3167 - 0.1e1 * t3287) * t2624 + t2083 - 0.1e1 * t2084) * t2626) * t2627 + t2889 * t2620) * t2618 + (-0.1e1 * t2314 * t2625 + (t2625 * t2783 + t2920) * t2621) * t2619 + (t2620 * t3904 + (-0.1e1 * t2201 * t2620 + t2626 * t2900) * t2621) * t2625 + (((t2626 * t4138 - 0.21751134959804000000000000000000e-1) * t2620 - 0.1e1 * t3069 + t3027) * t2618 + (t2619 * t3500 + t2719 + t2757) * t2625 + t4208) * t2628) * t2622;
  t1621 = t1666 * t3710;
  t1260 = (t1621 - t3508) * t2612 - t1508 + t3249 - t3965;
  t1302 = (-t1513 * t2618 + t3587) * t2626;
  t1368 = -0.1e1 * t3858 + t3851 + (-0.2e1 * t1668 + 0.62456754913197860000000000000000e-2) * t3832;
  t1788 = -t3252 + t3958;
  t1863 = 0.2e1 * t1963 * t3832;
  t2815 = t4027 - t3186 + (-0.2e1 * t1968 * t2625 - 0.1e1 * t1514) * t2618;
  t3008 = t2618 * (-0.2e1 * t1666 - 0.62456754913197860000000000000000e-2);
  t2959 = t2625 * t3008;
  t2671 = (((-t1643 + t3184) * t2626 + t4368 + ((0.2e1 * t3976 + 0.1e1 * t1513) * t2626 + t1841) * t2618) * t3842 + ((t1368 * t2612 + (t1801 - 0.1e1 * t4369) * t2626 + t1806 - 0.1e1 * t1809 * t2618 + t1863 + t3759) * t3784 + (-0.1e1 * t1624 * t2618 + (t2517 - t4315) * t2625) * t2626 - 0.2e1 * t2621 * t3476 - 0.1e1 * t1427 * t2618 - 0.1e1 * t1962 * t3792 + (t4027 - 0.1e1 * t3186) * t3818) * t2627 + ((-0.1e1 * t1608 * t2618 + t2625 * t3165) * t2626 - 0.1e1 * t1443 * t2618 - 0.1e1 * t1986 * t3792 + (t1545 * t2612 + t1875 * t2625 + (-0.1e1 * t3851 + t2959) * t3826) * t2621) * t2620 + t2815 * t3789 - t1583 * t2618 + t1551 * t3792 - t2625 * t3079) * t4064 + t1260 * t3630 + t1788 * t3593 + ((t1302 + t4370) * t2620 - t1771) * t3590 + (t1863 + t3293) * t3627 - t2629 * t3156;
  t1029 = -t2658 / 0.2e1 + t2671;
  t2727 = -0.13609823097337500000000000000000e-1 * t2619 + t4275;
  t2751 = (-0.1e1 * t3969 - t1936) * t2627 + (t2913 + t3345) * t2619;
  t2952 = -0.26431758938496000000000000000000e-1 * t2619 + t4014;
  t2778 = t2619 * t3146 + t2627 * t2952;
  t2921 = t2954 * t2627;
  t2659 = (((-0.56786982094425000000000000000000e-2 - t3962) * t2627 + t4157 * t2626 - t3952 + t3145) * t2618 + (t2626 * t4087 - 0.52129746651620000000000000000000e-1 * t2620 + t4227) * t2625 - t2953 * t2626) * t4067 + (t2751 * t2618 + t2778 * t2625 + t2619 * t2921 + (t2618 * t2727 - t3951) * t2620) * t4059;
  t1424 = t1549 * t2620 - t1986 * t2619;
  t1766 = -t1845 - t3233;
  t2963 = t3186 + t3769;
  t3065 = t2620 * t3188;
  t3067 = t2619 * t3188;
  t2682 = ((-0.1e1 * t4001 + t1302 + t3766) * t2613 + ((-0.1e1 * t1432 * t2618 - t3187) * t2626 - 0.1e1 * t1734 * t2618 + t1904) * t2627 + (-0.1e1 * t1416 * t2618 - t3065 + t2963) * t2626 - 0.1e1 * t1766 * t2618 - t1744 * t3798 + t1904 + (((t1621 + t3404) * t2612 + (-0.1e1 * t2024 * t3798 + t2509) * t2626 - 0.2e1 * t3700 - 0.1e1 * t3851 + t1881 - t3965) * t2627 + t1986 * t2625) * t2620) * t4066 + t1424 * t3624 + ((t3947 - t4016) * t2626 + t2815 * t2619) * t3595 + (-t1960 + t3067) * t3596 - 0.10875567479902000000000000000000e-1 * t2625 * t3785 + t1545 * t3465 + (t1968 * t3712 + t2959) * t3473 / 0.2e1;
  t1042 = -t2659 + t2682;
  t1099 = (t1880 + t3293) * t4075 + ((t1302 + t3252 + t2824 * t2625 + (-0.1e1 * t3028 * t2618 + t3020 * t2625) * t2619) * t2620 - t1771) * t4061 + t1260 * t4079 + t1788 * t4068 - t3156;
  t3127 = t1029 * t2637 + t1042 * t2636 + t1099 * t2635;
  t2950 = -0.988270895904e-3 * t2627 + t3435;
  t3081 = t2618 * t3166;
  t2996 = t2619 * t3081;
  t3082 = t2626 * t3254;
  t2997 = t2627 * t3082;
  t2657 = ((((-t2621 * t3172 + (-t2950 + 0.1200936784896e-2) * t2628) * t2625 + t2621 * t3341 - t3333 + t2896) * t2626 + (t3283 * t3415 + (-t2621 * t3426 + t2205) * t2619) * t2625 + (-t2619 * t3713 - t3338) * t2627 + (t2618 * t2897 - t2619 * t3423) * t2620 + t2619 * t3339 + t3338) * t2624 + ((((-t3422 + t3287) * t2627 + (-0.2970426191616e-2 + t3434) * t2628) * t2625 + t2621 * t3342 - t3334 - t2205) * t2626 + (-t2557 * t3415 + (t2519 + (0.2444413220184e-2 + t3425) * t2621) * t2619) * t2625 + (-t2619 * t2897 + t3337) * t2627 + (-t2618 * t3713 - t2619 * t3424) * t2620 + t2619 * t3340 - t3337) * t2617 + t2621 * t2997 + t2621 * t3066 + t2996) * t2622;
  t1299 = t2612 * t4124 + t1511 - t3907;
  t2666 = ((t2619 * t3501 + t4373) * t3842 + ((t1821 + t2976) * t3784 + ((-t2628 * t4222 + t3752) * t2625 - t1707 * t3819 + t3753) * t2626 + t2119 * t3830 + (t2114 * t2628 + (-t3719 + t4285) * t2621) * t2619) * t2627 + ((t2119 * t3792 - t3751) * t2626 + t3580 * t2625 + t3351 * t2628 + (-t3684 - t4334 + t4248 + (t2626 * t4286 + t3910) * t2619) * t2621) * t2620 + (t2114 * t2621 + (t3480 + t4036) * t2628) * t2626 + (t2621 * t4222 - t3911) * t3798 + (-t2112 * t2619 + t2618 * t4332) * t2628) * t4064 + (t1858 * t2605 - t4231) * t4058 + t1299 * t3630 + ((t2619 * t3718 - t1998 - t4373) * t2620 + t3757) * t3590 + (t3141 + t4145) * t3627 + t2629 * t3466;
  t1036 = -t2657 / 0.2e1 + t2666;
  t2795 = t2627 * t2901 - t3434;
  t3086 = t2618 * t3239;
  t2804 = -t2619 * t3172 - t3086;
  t3085 = t2618 * t3237;
  t2805 = -t2619 * t3173 + t3085;
  t2230 = -t2362 + t3705;
  t2903 = 0.7735484874e-2 * t2230 - t3190;
  t2904 = 0.3127439544e-2 * t2230 + t3191;
  t2906 = t3286 + t3454;
  t2911 = 0.7735484874e-2 * t3868 + 0.16724826617837780000000000000000e-2;
  t2912 = -0.3127439544e-2 * t3868 + 0.54835910640823200000000000000000e-3;
  t2566 = 0.316e0 * t2620 - 0.825e-1;
  t2960 = 0.7735484874e-2 * t2566 + t3427;
  t2961 = -0.3127439544e-2 * t2566 - t3428;
  t3017 = 0.988270895904e-3 - t3435;
  t2669 = ((t2617 * t2911 + t2624 * t2912) * t2626 + (t2617 * t2904 + t2624 * t2903) * t2619 + (t2617 * t2960 + t2624 * t2961 + t3243) * t2618) * t4067 + (((0.2444413220184e-2 + t2795) * t2626 + t3418 + t2805) * t2624 + ((t2627 * t2906 + t3017) * t2626 + t3419 + t2804) * t2617 + t2997 + t3066) * t4059;
  t2028 = t3719 * t2619;
  t2039 = t2119 * t2618;
  t2938 = (-0.1e1 * t1858 + t4124) * t2619 - t3724;
  t2684 = ((t1392 + t3588) * t2613 + (t3793 * t4222 - t2039) * t2627 + ((-t2040 + t3586) * t2625 + t3583) * t2626 - t2039 + (t3327 - t3918) * t2619 + ((-t3907 + t4112) * t2627 - t3351) * t2620) * t4066 + ((t2119 * t2619 + t1707) * t2620 + t4222 * t2619) * t3603 + (t2620 * t2938 + t2114) * t3601 + (t2619 * t4285 + t2626 * t3327 - t2028) * t3595 - t3597 * t4248 - t1524 * t3465;
  t1052 = -t2669 + t2684;
  t3078 = t2619 * t3206;
  t1105 = (-t2123 * t2617 - t3078 + t3141) * t4075 + ((t1392 - 0.1e1 * t1998 + (-0.1e1 * t1938 * t2617 + t2480) * t2618 + ((t2381 + (-0.13614453378240000000000000000000e-2 + t3261) * t2624) * t2618 - 0.1e1 * t3262 - 0.1e1 * t3194) * t2619) * t2620 - t3686 + t2617 * t3247 + t3078) * t4061 + t1299 * t4079 + t2605 * t2617 * t3200 - t2605 * t3276 - (-t2605 * t3269 + 0.13614453378240000000000000000000e-2) * t2617 / 0.2e1 + t2918;
  t3126 = t1036 * t2637 + t1052 * t2636 + t1105 * t2635;
  t3112 = t1192 * t3219;
  t3110 = t1192 * t3159;
  t3101 = t2618 * t3282;
  t3084 = t2618 * t3201;
  t3077 = t2619 * t3182;
  t3076 = t2620 * t2478;
  t3074 = t2620 * t3162;
  t3072 = t2621 * t3170;
  t3070 = t2626 * t2474;
  t3064 = t2625 * t3194;
  t3061 = t2625 * t3173;
  t3060 = t2625 * t3172;
  t3059 = t2625 * t3171;
  t3056 = t2628 * t2385;
  t3038 = t2626 * t4164 - t3914;
  t3025 = t2165 + t3216;
  t3021 = t2201 + t3214;
  t3014 = 0.2444413220184e-2 - t3434;
  t3006 = -0.1e1 * t3962 - 0.56786982094425000000000000000000e-2;
  t2995 = t3162 * t3787;
  t2993 = t2620 * t3082;
  t2992 = t2625 * t3074;
  t2183 = 0.82500000000000000000000000000000e-1 * t4298;
  t2303 = t2624 * t3174;
  t2975 = t2618 * (-t2183 * t3451 + t2303 - t3216);
  t2968 = -t3450 + t3451;
  t2964 = t1956 * t2625 + t3737 + 0.2e1 * t3975 + 0.26431758938496000000000000000000e-1;
  t2962 = (t2625 * t3586 + t3583) * t2619;
  t2677 = t1519 * t3472 + ((-0.1e1 * t1428 * t2619 + t3381 * t2626) * t2620 + (t1493 * t2612 - 0.1e1 * t3524 * t2619 + t1391 * t3789) * t2625 + (-0.1e1 * t1713 * t2619 + t1691 * t2626 + (t4235 * t2612 + (-0.2e1 * t3514 * t2626 + t4115 * t2619) * t2619) * t2628) * t2627 + ((t2358 * t2618 - t3320 + 0.3030488946654060e-2) * t2612 + t3004 * t2626 + ((-0.11357396418885000000000000000000e-1 + (t3383 - 0.1e1 * t2358) * t2619) * t2618 + (0.2e1 * t1444 - t3290 - 0.1580434873263008e-2 * t3838 + 0.12005987621373214000000000000000e-1) * t2626 - t2925) * t2619) * t2621) * t4065 + t2930 * t3617 + t2978 * t3600 + t1362 * t2612 * t3594;
  t2678 = (t2628 * t3132 + ((t3984 + (t1978 - t4024) * t2620) * t3789 + t3477 + (-t1962 * t3813 + (t2003 * t2628 + t3963) * t2620) * t2619) * t2625 + ((t2513 + t3355) * t2628 + t4159 * t2621) * t2626 + t3783 * t3988 + (t3072 + (t2628 * t4299 + t3223) * t2620) * t3835 + (t2621 * t4228 + t2628 * t3506) * t2619 + t2627 * t3164) * t4064 - 0.11563098993883908500000000000000e-1 * t3782 + (t2618 * t3716 + t3715) * t3599 + ((-t1903 + t3770) * t2626 + t3409) * t3591 + t1603 * t3628 + (t1909 + t3970) * t3617 + t2629 * t3468 + t3459 * t4013;
  t1034 = t2677 + t2678;
  t2683 = (-0.1e1 * t1519 * t2605 - 0.1e1 * ((-0.1e1 * t3964 + t2770) * t2625 - 0.1e1 * t3890 + t2865) * t2619 + (0.2e1 * t2619 * t3134 + t3052 * t4082 + t2869) * t2626) * t4060 + (t1519 * t2627 * t3709 - t2605 * t2887 - t2619 * t2777 + t2626 * t2746) * t4067;
  t2125 = t3170 + t3233;
  t2691 = ((t2303 - t3982 + t4192) * t2626 + (t2125 * t2618 + t4228) * t2619) * t4059 + (-0.1e1 * t3692 * t2611 + (t3756 * t2626 - 0.1e1 * t1871 + (-0.1e1 * t4252 - 0.1e1 * t3952) * t2620) * t2625 + (-t2513 - 0.1e1 * t3355) * t2626 + t3443 * t3823 + (-t1971 * t2611 + (-0.1e1 * t3216 - 0.1e1 * t2165) * t2619 + t4088) * t2627) * t4066 + (t3756 + t3964) * t2625 * t3598;
  t1057 = t2683 + t2691;
  t1500 = t2017 * t2618 + t2987;
  t2893 = t1531 + t3951;
  t2695 = ((-t3303 + t4163) * t3709 + t4111 * t2612 - (t2619 * t4111 + t3044) * t2619 + t1962 * t3793 - t3886) * t4069 + t1833 * t3602 + t2893 * t3618 + t1500 * t2627 * t3605 + t2626 * t3467;
  t1403 = t2619 * t3021 + t4252;
  t2701 = (t2619 * t3025 + 0.23126197987767817000000000000000e-1) * t4069 + (t1403 * t2625 + t3511 * t2626 + (t4317 + t2474 - 0.1e1 * t2158) * t2619) * t4061 + (t2460 * t2618 - t3238) * t4062 + t3468 - t1971 * t3849 / 0.2e1 + (-t1962 * t2626 - t3975) * t3607;
  t1078 = t2695 + t2701;
  t1799 = t2274 + t3303;
  t1176 = (t1799 * t2626 - t1702 + t1989) * t3175 + ((-0.36699518879455040000000000000000e-2 + t3768 - 0.1e1 * t4150) * t2626 - 0.1e1 * t1799 * t3241) * t2619 + ((-t3047 + 0.1e1 * t4010) * t2625 + t2171) * t3241;
  t2634 = q_state_dot(4);
  t2948 = -t1034 * t2637 - t1057 * t2636 - t1078 * t2635 + t1176 * t2634;
  t2665 = ((-0.1e1 * (t2130 * t3800 + (t2182 * t2626 - 0.56786982094425000000000000000000e-2) * t2621) * t2620 + t2870 * t2627 + ((-0.1e1 * t3984 - 0.1e1 * t3968) * t2619 - 0.1e1 * t2201 * t3791 - t2883 * t2627) * t2628) * t2618 + (-t2124 * t3792 + t2953 * t3784) * t2619 + (-(t2621 * t2862 + t4097) * t2620 + (t2621 * t2863 + t3350) * t2627) * t2625) * t4064 + (-t2003 * t2620 + t2627 * t2759) * t3591 + (t2625 * t3716 + t2921) * t3617 + (t2619 * t3356 + t2627 * t2837 - t4316) * t3622;
  t1831 = t2627 * t3690;
  t2308 = t2624 * t3191;
  t1879 = t2236 * t2625 + t2308;
  t2936 = t4138 * t3797;
  t2670 = (t4364 * t4257 + ((-t1831 - 0.1e1 * t1493 * t2618) * t2619 - 0.1e1 * t1377 * t2618 + t1656 * t3784 + (t3008 * t3655 + (-t2125 + t2866) * t2621) * t2625) * t2626 + (t1667 * t3710 + t3508) * t3852 + (-0.1e1 * t1391 * t2618 + (t2620 * t2964 + t3170) * t2625) * t3785 - t1510 * t2618 + ((-t3214 - 0.1e1 * t2236) * t3792 - t2625 * t3073 + t2182 * t3796) * t2627 + t2621 * t2936 - t2621 * t3064 - t2177 * t3796) * t4064 + t1879 * t3593 + (t1368 * t3823 + (t1656 - t3947) * t2627) * t3599 + (-0.1e1 * t1388 * t2618 - t3065 + t2964 * t3786) * t3617 - t3594 * t4317 - t4364 * t3464;
  t1040 = -t2665 + t2670;
  t2668 = ((-0.1e1 * t3006 * t2620 + t2302 * t2626) * t2618 - 0.1e1 * t2768 * t3797) * t4059 + ((-0.1e1 * (-0.1e1 * t1936 - 0.1e1 * t3969) * t2620 + t1962 * t3825) * t2618 - 0.1e1 * t2952 * t3797 - 0.1e1 * t2619 * t2922) * t4066 + ((t4198 * t2618 + (-0.1e1 * t1986 - 0.1e1 * t3177) * t2625) * t4059 + (t4275 * t2618 + (-0.1e1 * t2003 + t3242) * t2625) * t4066) * t2627;
  t2888 = t4275 * t2625;
  t2675 = ((t1378 * t3790 - t3984 * t2618 + t1968 * t3527 - t3058 + ((t3005 + t3892) * t2611 - t1499 * t2618 - t3186) * t2620) * t2619 - t4364 * t3845 + (t2025 * t3834 + t2620 * t2888) * t2626 + t4313 + t1879 * t2627) * t4066 + ((t1697 * t3710 + t3508) * t2605 - t4364 * t3826 + (-t2618 * t2753 - t2620 * t3187 + t2509 - t3058) * t2626 - t2781 * t2618 + t3022 * t3786 + t2936 - t3064 - t3885) * t4059;
  t1061 = -t2668 + t2675;
  t2808 = t2981 - t3186;
  t2789 = -0.1e1 * t1978 * t2618 - t3892 + t2808;
  t2697 = (t2789 * t2619 + (-0.1e1 * t3836 + (-t2390 + t3500) * t2625) * t2626) * t4061 + ((-t2079 - t3076) * t2618 + t3065) * t4070 + t2201 * t3608 + t3463 - t3240 * t3794;
  t2699 = t1797 + 0.13215879469248000000000000000000e-1 * t2619 * t3786 + (-t4363 * t2612 + (t1870 + (-0.1e1 * t3858 + (-0.2e1 * t1696 + 0.6245675491319786e-2) * t3832) * t2619) * t2626 + t1549 * t2618 - t3067 + t2308 + t2201 * t2625) * t4068 + (t1656 - t3836) * t3602 + t1500 * t2618 * t3619 + (t2017 * t2625 + t3737) * t3461;
  t1093 = -t2697 + t2699;
  t1213 = t1404 * t4080 + t4363 * t3620 + (0.1e1 * t3047 * t2626 - 0.52863517876992000000000000000000e-1) * t4071 + 0.50000000000000000000000000000000e0 * t3885 + (-0.1e1 * t3177 + t2469) * t2625;
  t2947 = t1040 * t2637 + t1061 * t2636 + t1093 * t2635 + t1213 * t2634;
  t2651 = t2992 + t2626 * t2995 + ((((t2205 * t2620 - t2621 * t3428) * t2625 + (t2620 * t3453 + t3427) * t2628) * t2626 + (-t3283 * t3531 - 0.1200936784896e-2 * t3823) * t3792 - t2868 * t2620 + t2787 * t2627) * t2624 + (((-(-t3285 - t3431) * t2620 + t2621 * t3427) * t2625 + t2620 * t3340 + t2627 * t3424) * t2626 + (t2557 * t3531 + 0.2970426191616e-2 * t3823) * t3792 - t3013 * t2620 + t2786 * t2627) * t2617 + t2628 * t2993 - t2625 * t3057) * t4064 + ((t2627 * t2902 - t3435) * t2626 + (-t2557 * t2620 + 0.4038528e-2 * t3825) * t3535 + t2804) * t3626 + (t2795 * t2626 + (t2620 * t3283 - 0.1632768e-2 * t3825) * t3535 + t2805) * t3609;
  t2656 = t4248 * t3594 + (-0.1e1 * t2040 * t2625 + (t3719 + t3361) * t2627) * t3617 + (t3377 + (t1414 * t2619 + t3724) * t2620) * t3599 - 0.1e1 * t1707 * t3460 + t1524 * t3464 + (((t3754 - 0.1e1 * t3911) * t2625 + t1522 * t2628) * t3791 + t1525 * t3852 + (-0.1e1 * t3751 * t2627 + (-0.1e1 * t2617 * t3229 - 0.1e1 * t3073) * t2620 + t2287 + (t4170 + (0.1e1 * t3719 + t3361) * t2620) * t2628) * t2619 + t2628 * t4335 + (t2626 * t2938 - t4362) * t3783 + ((-0.1e1 * t3122 + 0.790217436631504e-3 * t4276) * t2612 + (((0.4841887557042460e-2 * t2610 - 0.1e1 * t2234 * t2617 + t3749) * t2625 + 0.1096718212816464e-2 * t3840 - 0.3344965323567556e-2 * t2618 * t2624) * t2619 + (-0.1e1 * t3909 - 0.1e1 * t2111) * t2625) * t2626 + t3271 * t2619 - 0.1e1 * t3084 - 0.1e1 * t2479 + t4323) * t2621) * t4064;
  t1044 = -t2651 + t2656;
  t2667 = (((0.6381775021050e-3 * t2617 - 0.2580137623800e-3 * t2624) * t2627 + (0.2444413220184e-2 * t2617 - 0.988270895904e-3 * t2624) * t2620) * t3793 + ((-0.2444413220184e-2 * t2620 - t3427) * t2624 + (-t3428 - t4101) * t2617) * t2619 + (t2617 * t2949 + t2624 * t2950) * t2618) * t4059 + ((t4103 * t2626 + (t2627 * t3283 + t3388) * t3535 + t2807) * t2624 + ((-t2620 * t2906 - t3428) * t2626 + (-t3387 - t2351) * t3535 + t2806) * t2617 - t2993 + t3059) * t4066;
  t2882 = -0.68072266891200000000000000000000e-3 + t3265;
  t2679 = ((t1414 * t3790 - t4170 + ((-0.1e1 * t4264 - 0.1e1 * t3926 + t4209) * t2625 + t3480) * t2620) * t2619 + t1524 * t3845 + (t2030 + (t4247 - t4205) * t2620 + (-t2624 * t2882 - t2385) * t3834) * t2626 - t1707 * t3786 - t4335) * t4066 + (t1525 * t2605 + (-t2114 * t2620 - t2030 - t4358) * t2619 - t1822 + (t2620 * t4222 - t2111 - t3909) * t3793 - t3084 - t2479 + t4323) * t4059;
  t1071 = -t2667 + t2679;
  t2773 = t2568 * t2967 + t3254 + t4247;
  t2692 = t3212 * t3834 + 0.36776100000000000000000000000000e0 * (-0.8676525e-3 * t2624 - 0.3507900e-3 * t2617) * t3791 + (t2098 * t3077 - 0.1e1 * t2617 * t3244 - 0.1e1 * t2619 * t3214 + t2626 * t2773) * t4061 - 0.1e1 * t3240 * t3840 + (-0.735522e0 * t2557 * t2617 + t2624 * t4206 + 0.49096519673609460000000000000000e-2) * t3607;
  t2703 = (t3724 * t2626 - t2617 * t3256 + t2618 * t3203 + (t1414 * t2626 - t3910) * t2619 + t4362) * t4068 - t3719 * t3619 + t3377 * t4062 + t3618 * t2027 + (t3326 + t3926) * t3461;
  t1102 = -t2692 + t2703;
  t1207 = t4358 * t3241 - 0.38677424370000000000000000000000e-2 * t2168 * t2617 + (0.12009367848960000000000000000000e-2 * t2618 + 0.27521467987200000000000000000000e-3) * t2624 + t1865 * t4094 + 0.50000000000000000000000000000000e0 * t2605 * t4124 + 0.50000000000000000000000000000000e0 * t3686;
  t2946 = t1044 * t2637 + t1071 * t2636 + t1102 * t2635 + t1207 * t2634;
  t2940 = t2990 * t2618;
  t2934 = -0.1200936784896e-2 * t2625 - 0.54835910640823200000000000000000e-3;
  t2933 = 0.2970426191616e-2 * t2625 - 0.16724826617837780000000000000000e-2;
  t2899 = t3256 - t3442;
  t2898 = 0.16724826617837780000000000000000e-2 * t2618 + t3441;
  t2660 = ((t2915 * t2626 - 0.1e1 * t3124 * t3825 + ((-0.1e1 * t2478 - 0.1e1 * t4089) * t3817 + t2286) * t2619) * t2618 + t2732 * t2626 + (t2628 * t2900 + t2765) * t3798 - 0.1e1 * t2162 * t2619 * t3816 + (t4258 - 0.1e1 * t2386 - 0.1e1 * t3043) * t3818) * t4065 + t2861 * t3600 + (t2626 * t2752 - t2867 * t3823) * t3623 + t2772 * t3372;
  t2696 = t2629 * t3478 - t3315 * t2618 * t3780 + (-t3125 * t2618 + (-0.2e1 * t2916 * t2618 + t1509 * t2626 + t3698 * t4083 + t1495 * t2619 + (t1697 * t3640 + t1469) * t2625) * t2625) * t4064 + (t1694 * t3791 + t1968 * t2627) * t3628 + t3138 * t3623 + t1983 * t2626 * t3591 + t1744 * t3372;
  t1046 = t2660 + t2696;
  t2686 = ((-t1936 + (t1932 - t4157) * t2619) * t2618 + (t2619 * t2782 + t4014) * t2625 + t2953 * t2619) * t4060 + (((-t1978 * t2626 + t3952) * t2627 + (t2176 * t2967 - t3234 + 0.52129746651620000000000000000000e-1) * t2626) * t2618 + ((-t1720 - t3176) * t2627 + t3146 * t2626) * t2625 + t2626 * t2921) * t4067;
  t2711 = -t2628 * t3476 + (-t1281 * t2618 + (t1744 * t3825 + t2783 * t2626 + (t1694 * t3790 - t1968 * t2620) * t2625 + (t1887 * t2620 - t1603) * t4083) * t2625) * t4066 + t1321 * t3624 + (t1984 * t2619 - t4014) * t3603 + t3598 * t1661;
  t1068 = t2686 + t2711;
  t2790 = t2183 * t3449 + t2080 - t4089;
  t2698 = (t2789 * t2626 + (t2888 + t3836) * t2619) * t4068 + (t2618 * t2790 - t3058 + t3188) * t4062;
  t2714 = t3478 - t1971 * t3662 + (t3703 - 0.1e1 * t1403 * t2618 + (t1720 + (-0.2e1 * t3975 - 0.26431758938496000000000000000000e-1) * t2626) * t2625) * t4068 + (t1686 * t2626 + t1871) * t4071 + t3467 + t2174 * t3793 / 0.2e1;
  t1106 = -t2698 + t2714;
  t1165 = -0.1e1 * (t2981 + t4119) * t3241 + t2003 * t3831 - 0.1e1 * (-0.1e1 * t2940 + t3769) * t3241 - 0.10000000000000000000000000000000e1 * t1744 * t3793;
  t1383 = t3851 / 0.2e1 - t3858 / 0.2e1 + (t1945 - t1971) * t3832;
  t2633 = q_state_dot(5);
  t2892 = t1046 * t2637 + t1068 * t2636 + t1106 * t2635 - t1165 * t2634 + t1383 * t2633;
  t2653 = ((-t2731 * t2619 + (-t3228 + (t3016 - t3435) * t2628) * t3793 + t2896 * t3790) * t2624 + (-t2710 * t2619 + ((-t3425 + t3434) * t2628 + t3713) * t3793 - t2205 * t3790) * t2617 + t2627 * t2996 + t2621 * t3082 + ((-t3333 + t3343) * t2624 + (-t3334 + t3344) * t2617) * t2626) * t4064 + (-t2764 * t2619 + (t3139 + t3489) * t3412 - t2620 * t3178) * t3626 + (-t2763 * t2619 + (-t3140 - t3490) * t3412 - t2620 * t3179) * t3609 - t3074 * t3835;
  t2797 = -t2102 * t3787 + t2626 * t4304;
  t2663 = ((t2102 * t3310 - t3784 * t4231) * t2611 + (((-t2040 + (t1673 - 0.1e1 * t2103) * t2627 - t4222) * t2628 + t3752) * t2626 + (t1710 * t3818 - t2102 * t3784) * t2618 + (t2852 * t3783 + (t2040 + t3924) * t2621 + t3755) * t2619) * t2625 + (((t2159 - t3204) * t2617 + t2854) * t3819 + t3719 * t3783 + t2114 * t3813 - t3724 * t3817 + t3753) * t2626 - t2628 * t3654 - t3637 * t4319 + ((t2112 * t2627 - t2620 * t3724 + t2114) * t2628 - t3719 * t2621) * t2619) * t4064 + (t2620 * t3038 + t2797) * t3591 + (-t2102 * t3791 - t2627 * t4231) * t3628 + (-t2112 * t2620 - t2030 + t3724) * t3617 + t2629 * t3469 - t3593 * t3922 + t1707 * t2620 * t3459;
  t1058 = -t2653 + t2663;
  t2681 = ((-0.1e1 * t3014 * t2619 - t3448 * t4191) * t2624 + (-0.1e1 * t3017 * t2619 + t3447 * t4191) * t2617 + ((-0.1e1 * t2901 * t2619 - t3179) * t2624 + (-0.1e1 * t2906 * t2619 - t3178) * t2617 - t2618 * t3243) * t2627) * t4066 + ((-0.1e1 * t2912 * t2619 + t2903 * t2626) * t2624 + (-0.1e1 * t2911 * t2619 + t2904 * t2626) * t2617 + t3082) * t4059;
  t2285 = t2620 * t3216;
  t2688 = ((-t4320 + t2469 - t3076 + t3346 + t3918) * t2626 - t2028) * t4059 + ((-0.1e1 * t2102 * t3790 + t4231 * t2620) * t2611 + ((t2176 * t3451 + t2285 - t3211) * t2626 + t2102 * t3834 + t3038 * t2627) * t2625 - t3719 * t3790 + (-t3345 + t3076 - t3199 + (t4320 - 0.1e1 * t2112) * t2627) * t2619 + t3654) * t4066 + (t3912 + (t2175 * t3451 + t1677 + t2285 - t2474 + t3924) * t2619) * t3603 - t2102 * t3674 / 0.2e1;
  t1086 = -t2681 + t2688;
  t2690 = 0.12900688119000000000000000000000e-3 * t3839 + 0.31908875105250000000000000000000e-3 * t3827 + t2797 * t4063 + (t1707 * t3835 - t2102 * t3848 + t2619 * t4284 + t3793 * t4164 - t3922) * t4068 + t3469 - t4231 * t3629 - t3724 * t3618;
  t2694 = (t3182 * t2038 - 0.1e1 * t2617 * t3178 - 0.1e1 * t2619 * t2773 - 0.1e1 * t2624 * t3179) * t4068 + 0.36776100000000000000000000000000e0 * t2565 * t3860 + (t2617 * t3139 - t2624 * t3140) * t4063 * t3534;
  t1135 = t2690 - t2694;
  t2784 = -0.34036133445600000000000000000000e-3 * t2624 - 0.13760733993600000000000000000000e-3 * t2617 - 0.24548259836804730000000000000000e-2;
  t2853 = -0.27417955320411600000000000000000e-3 * t2617 + t3212;
  t2878 = t2933 * t3839;
  t2879 = t2934 * t3827;
  t1198 = (0.14852130958080000000000000000000e-2 * t2624 + 0.60046839244800000000000000000000e-3 * t2617 + (-0.1e1 * t2853 - 0.1e1 * t3280) * t2625 + (-0.1e1 * t2784 + t3282) * t2618) * t2626 - 0.1e1 * t2112 * t3175 + 0.50000000000000000000000000000000e0 * t2962 + 0.50000000000000000000000000000000e0 * t2879 + 0.50000000000000000000000000000000e0 * t2878;
  t1501 = t3631 - t3665 / 0.2e1 - t4231 * t2611 / 0.2e1;
  t2891 = t1058 * t2637 + t1086 * t2636 + t1135 * t2635 + t1198 * t2634 + t1501 * t2633;
  t2873 = t2626 * t2898;
  t2654 = t2995 + t2626 * t2992 + (((-t2618 * t2877 - t3441 * t3783) * t2626 - t2748 * t2618 - t2627 * t3332 + t2205 * t3797 + t3441 * t3818 + t3332) * t2624 + ((-t2618 * t2754 - t3442 * t3783) * t2626 - t2816 * t2618 + t2627 * t3331 + t2896 * t3797 + t3442 * t3818 - t3331) * t2617 + t2620 * t3081 + t4131 * t2625) * t4064 + (-t2618 * t2945 - t2899 * t3791 + t3061) * t3626 + (-t2618 * t2944 + t2620 * t2873 - t3060) * t3609;
  t2316 = t2628 * t3211;
  t2661 = ((-0.1e1 * t2103 * t2620 - t4304) * t2619 + t1707 * t2627 + (0.5483591064082320000000000000000e-3 * t2617 - 0.1e1 * t3203) * t3791) * t3622 + (t1707 * t3791 - 0.1e1 * t2852 * t2627) * t3591 + t1705 * t2619 * t3593 + (((-0.1e1 * t2126 * t2617 - 0.1e1 * t2294 - 0.1e1 * t2316 + (t2103 * t2627 + t2040) * t2628) * t2619 + (-0.1e1 * t2130 * t2617 + (t2518 - 0.1e1 * t3229) * t2624) * t3790 + (t3056 - 0.1e1 * t1844 * t2617 + (t2621 * t3180 + t2628 * t2882) * t2624) * t2620 + t2626 * t2240 - 0.1e1 * t2621 * t3070) * t2618 + ((-0.1e1 * t2621 * t3898 + t3580) * t2625 + t1710 * t3783) * t2619 + ((-0.1e1 * t2626 * t3056 - 0.1e1 * t1861 * t2617) * t2627 + (-0.1e1 * t2127 * t2617 - 0.1e1 * t2292) * t2620 + (-0.1e1 * t2621 * t3174 + (-0.1e1 * t2882 * t3790 + t3237) * t2628) * t2624 + t3750) * t2625 + t2626 * t3097 + (-0.1e1 * t3089 - 0.1e1 * t3893 - 0.1e1 * t2026) * t3815) * t4064;
  t1063 = -t2654 + t2661;
  t2685 = (((t2362 * t3448 + t3244) * t2624 + (-t2362 * t3447 - t3246) * t2617) * t2618 + ((0.680722668912e-3 * t2619 + t2961) * t2624 + (0.275214679872e-3 * t2619 + t2960) * t2617 + t3243) * t2625) * t4059 + ((-t2066 * t3541 + t2620 * t3190 + t2627 * t2873) * t2624 + ((-0.5483591064082320000000000000000e-3 * t2618 + t3442) * t3790 - t2060 * t3541 - t2620 * t3191) * t2617 + t2626 * t3059 - t2620 * t3254) * t4066;
  t2689 = ((t2175 * t2626 * t2968 + t3790 * t4222 + t3914) * t2618 + (-t2173 * t2968 - t3909 + t4319) * t2625 + t1710 * t2626) * t4060 + (((-t2103 * t2619 + t3912) * t2627 - t2968 * t2176 * t2619) * t2618 + t3790 * t4196 + t1705 * t3825 + (t4247 - t4320) * t2620) * t4067;
  t1096 = t2685 + t2689;
  t2831 = 0.680722668912e-3 * t2624 + 0.275214679872e-3 * t2617 + 0.49096519673609460000000000000000e-2;
  t2705 = ((-0.28244044800000000000000000000000e0 * t2037 - t3912) * t2618 + t2831 * t3793) * t4068 + (t2617 * t3379 + t2624 * t3378 - t3171) * t4071;
  t1153 = ((-0.1e1 * t2103 * t2618 + t1705) * t2619 + t2852 * t3831 + t2625 * t3095 - 0.1e1 * t2626 * t3684 + (t2249 - 0.1e1 * t2477) * t3793) * t4068 + t2975 * t4070 + t2627 * t3632 - t2617 * t3061 + t2624 * t3060 - t2705;
  t2704 = (t2617 * t2899 - t2624 * t2898 - t3189) * t4070 + (-t3430 + 0.1200936784896e-2 * t3831) * t2624 / 0.2e1 + (t3429 - 0.2970426191616e-2 * t3831) * t2617 / 0.2e1;
  t2716 = (t2618 * t2474 + (t3195 - 0.1e1 * t1965) * t2617 + t3018) * t4062 - t4332 * t4063 - t2852 * t3835 / 0.2e1;
  t1238 = -t2704 + t2716;
  t1375 = (t2853 - t3280) * t2625 + (t2784 + t3282) * t2618;
  t1698 = -t3276 + t3215 + (0.50000000000000000000000000000000e0 * t2162 + t3200) * t2617;
  t2632 = q_state_dot(6);
  t2846 = -t1063 * t2637 + t1096 * t2636 - t1153 * t2635 - t1238 * t2634 - t1375 * t2633 - t1698 * t2632;
  t2821 = -0.275214679872e-3 * t2618 - t3191 - 0.1200936784896e-2;
  t2820 = -0.680722668912e-3 * t2618 + t3190 - 0.2970426191616e-2;
  t2631 = q_state_dot(7);
  t2601 = 0.316e0 * t2629;
  t2143 = t3561 + t4253;
  t1376 = t2831 * t2618 / 0.2e1 + t4247 / 0.2e1 + t3101 + t2853 * t2625;
  t1239 = t2704 + t2716;
  t1199 = (t2617 * t2821 + t2624 * t2820 - t3254) * t4062 - t2879 / 0.2e1 - t2878 / 0.2e1 + t2962 / 0.2e1 + (-t4247 / 0.2e1 + t3632 - t2112 / 0.2e1) * t2626;
  t1185 = -(t2808 + t4119) * t2619 / 0.2e1 + (-t2940 + t2963) * t4070;
  t1162 = t2627 * t3101 + ((-0.1e1 * t2103 * t2618 - t1710) * t2620 + t2975) * t3241 + (t4248 + ((t3204 - 0.1e1 * t2159) * t2617 - t2854) * t2625) * t2620 * t3175 + t2705;
  t1136 = t2690 + t2694;
  t1107 = t2698 + t2714;
  t1103 = t2692 + t2703;
  t1095 = t2685 - t2689;
  t1094 = t2697 + t2699;
  t1087 = t2681 + t2688;
  t1080 = -0.74457943965523448900000000000000e0 + t1157 * t2613 + t1201 * t2627 + t1360 * t2612 + t1507 * t3826 + 0.18916511922000000000000000000000e0 * t2620 - t3748 + t4215;
  t1077 = -t2695 + t2701;
  t1072 = t2667 + t2679;
  t1069 = -t2686 + t2711;
  t1064 = t2654 + t2661;
  t1062 = t2668 + t2675;
  t1059 = t2653 + t2663;
  t1056 = -t2683 + t2691;
  t1053 = t2669 + t2684;
  t1051 = t1073 * t2628 - 0.796671776787104e-2 + (t2620 * t4236 + t2809) * t2621;
  t1048 = t1074 * t2614 + t1108 * t3812 + t1752 * t2627 + t1460 * t2626 + t1816 * t2620 + t3957 + 0.21165494803694631600000000000000e0;
  t1047 = -t2660 + t2696;
  t1045 = t2651 + t2656;
  t1043 = t2659 + t2682;
  t1041 = t2665 + t2670;
  t1038 = -t2673 + t2718;
  t1037 = t2657 / 0.2e1 + t2666;
  t1033 = -t2677 + t2678;
  t1032 = t2664 + t2700;
  t1030 = t2658 / 0.2e1 + t2671;
  t1028 = t2662 / 0.2e1 + t2672;
  t1022 = t2655 - t2687;
  t1015 = t2647 + t2650;
  t1013 = t2648 + t2652;
  t1011 = (t1048 - t1080) * t3805 + (-t2608 / 0.2e1 + t4072) * t1051;
  t1010 = t2649 + t2674;
  t1008 = -t2645 + t2676;
  t1006 = -t2646 + t2680;
  C(7,3) = -t1102 * t2634 - t1135 * t2633 - t1153 * t2632 - t3126;
  C(4,1) = t1007 * t2636 + t1023 * t2635 - t1034 * t2633 + t1040 * t2632 + t1044 * t2631 - t4057;
  C(6,3) = -t1093 * t2634 - t1106 * t2633 + t1153 * t2631 - t3127;
  C(1,1) = t1011 * t2636 + t1017 * t2634 + t1019 * t2633 + t1020 * t2632 + t1021 * t2635 + t1025 * t2631;
  C(5,4) = -t1165 * t2632 + t1198 * t2631 - t2948;
  C(7,5) = -t1375 * t2632 - t2891;
  C(3,7) = (((-t2568 * t2968 - t2625 * t3719) * t2626 + t2128 * t3077 + t2617 * t3246 - t2619 * t3203) * t2620 + 0.735522e0 * t2565 * t4245 + (-t2617 * t3378 + t2624 * t3379) * t2625 + t2617 * t3062 + t2624 * t3063) * t2631 + t1162 * t2632 + t1136 * t2633 + t1103 * t2634 + t3126;
  C(5,6) = t1376 * t2631 + (-t2275 - t3880 + t4016) * t2632 + t2892;
  C(5,1) = -t1009 * t2636 - t1027 * t2635 + t1034 * t2634 + t1046 * t2632 + t1058 * t2631 - t4056;
  C(2,5) = t1087 * t2631 + t1069 * t2632 + (((t2003 * t3786 + t1361) * t2626 + (-t1353 * t2625 - t1968 * t3847 - t1562) * t2619) * t2621 + ((-t1363 + t3951) * t2619 + (t1356 * t2625 + t1574 + t3851) * t2626) * t2628) * t2633 + t1056 * t2634 + t1038 * t2635 + t3366;
  C(2,3) = t1053 * t2631 + t1043 * t2632 + t1038 * t2633 + t1032 * t2634 + ((t1144 * t2627 + t1209 * t2613 + t1605 * t2620 + t1766 * t2625 + t2619 * t2989 + t2626 * t2747 + t1902 - 0.36044563611157510600000000000000e0) * t2628 - t1245 * t3813 - t1529 * t3673 - t2794 * t3815 - t1424 * t3796 - t1717 * t3817 + t2170 * t3818 + t3224) * t2635 + t3368;
  C(4,4) = t1176 * t2633 + t1207 * t2631 + t1213 * t2632;
  C(1,5) = t1059 * t2631 + t1047 * t2632 + (((t3655 + t3815) * t3851 + (-t1316 * t2619 + (t1694 * t3819 + t1374) * t2626) * t2625 - t2733 * t2619 + t1495 * t3831 + t2717 * t2626) * t2622 - t2629 * t1968 * t3675 + (-t1357 * t2619 + t2003 * t3791) * t3780 - t2905 * t3824 + t3639 * t4317 + t2917 * t3788) * t2633 + t1033 * t2634 + t1028 * t2635 + t1010 * t2636 + t4056;
  C(4,6) = t1239 * t2631 + ((t2451 - t4337) * t2626 - (t1962 - t1720) * t2618 + t2003 * t3798 - t3188) * t2632 + t1185 * t2633 + t2947;
  C(6,5) = t1375 * t2631 - t2892;
  C(7,4) = -t1198 * t2633 - t1238 * t2632 - t2946;
  C(5,7) = ((0.680722668912e-3 * t2617 - 0.275214679872e-3 * t2624) * t2625 - t3719 * t2618) * t2631 + t1376 * t2632 + t2891;
  C(7,7) = 0.0e0;
  C(6,7) = t2631 * t2852 - t2846;
  C(1,6) = t1064 * t2631 + ((((-0.1e1 * t1962 * t3784 + t1978 * t3783 + t3403) * t2619 + (t3509 - t3883) * t2620 + t3349 * t3790 + (0.56786982094425000000000000000000e-2 + (t2182 * t2627 + t2079 + t3007) * t2626 - t2125) * t2621) * t2625 + (-0.1e1 * t2894 * t2619 - 0.1e1 * t2802 - 0.1e1 * t3296 + (t2883 * t2619 - 0.1e1 * t2829 - 0.1e1 * t2830 - 0.1e1 * t2423 - t2780) * t2621) * t2618) * t2622 + t2712 * t3780 - t3824 * t3967 - t2743 * t3829) * t2632 + t1047 * t2633 + t1041 * t2634 + t1030 * t2635 + t1013 * t2636 + t4055;
  C(3,4) = t1103 * t2631 + t1094 * t2632 + t1077 * t2633 + (((-t2274 - 0.1e1 * t3900 + t4099) * t2612 + t4343 - t4348 + t3880 + t3382) * t2627 + (-0.1e1 * t2893 * t2626 + 0.1644487577369270e-2) * t2620 + ((t4111 * t2626 - 0.1e1 * t2172) * t2627 + (-0.1e1 * t1500 * t2625 + t3511) * t2620) * t2619) * t2634 + t3129;
  C(2,2) = -0.1e1 * t1035 * t2631 + t1026 * t2632 + t1024 * t2633 + t1018 * t2634 + t1016 * t2635 + t4177 - t4134 * t4177;
  C(2,7) = ((-0.1e1 * (t2626 * t3014 + t3085 + t3418) * t2617 + (t2626 * t3017 - t3086 + t3419) * t2624 + (-0.1e1 * (t2626 * t2901 - t3246) * t2617 + (t2626 * t2906 - t3244) * t2624) * t2627) * t2621 + ((-0.1e1 * t2912 * t2617 + t2911 * t2624) * t2626 + (-0.1e1 * t2903 * t2617 + t2904 * t2624) * t2619 + (-0.1e1 * t2961 * t2617 + t2960 * t2624) * t2618) * t2628) * t2631 + t1095 * t2632 + t1087 * t2633 + t1072 * t2634 + t1053 * t2635 + t3364;
  C(7,2) = -t1052 * t2635 - t1071 * t2634 - t1086 * t2633 + t1096 * t2632 - t3364;
  C(1,3) = t1037 * t2631 + t1030 * t2632 + t1028 * t2633 + t1022 * t2634 + (t2890 * t3843 + (-t1155 * t3817 + ((-0.1e1 * t3963 - 0.1e1 * t3946) * t2625 - 0.1e1 * t3889 - t1744 * t3830 - 0.1e1 * t3055 + t4193) * t2626 + t1968 * t3674 + (t1514 * t3785 + t3225) * t2625 - t1604 * t2621 - t3163 * t3835 - t1970 * t3785 + 0.1644487577369270e-2 * t2628) * t2627 + ((t2315 + (t1904 - 0.1e1 * t2172) * t2621) * t2626 + (-0.1e1 * t3223 - t2314) * t2625 + t1605 * t2621 + t1875 * t3830 + ((t2619 * t2857 + t2165) * t2626 + (t2814 + t3897) * t2625 - 0.1e1 * t3245 + t4098) * t2628) * t2620 + (-t2316 + t2881 * t2628 + (-0.1e1 * t3851 - 0.1e1 * t4043 - 0.1e1 * t1833) * t2621) * t2626 + (-t1845 * t2621 - t1986 * t3785) * t2625 - t1411 * t2621 - t2517 * t3835 + 0.46305794820080000000000000000000e-2 * t3785 - 0.13297019103287584000000000000000e-1 * t2628) * t2622 * t2635 + t1006 * t2636 + t4054;
  C(5,2) = t1039 * t2635 + t1057 * t2634 + t1068 * t2632 + t1086 * t2631 - t3366;
  C(3,2) = t1031 * t2634 - t1039 * t2633 + t1042 * t2632 + t1052 * t2631 - t3368;
  C(5,5) = t1383 * t2632 + t1501 * t2631;
  C(3,1) = t1005 * t2636 - t1023 * t2634 + t1027 * t2633 + t1029 * t2632 + t1036 * t2631 - t4054;
  C(3,5) = t1136 * t2631 + t1107 * t2632 + ((-t1870 + (-0.1e1 * t4166 * t2619 + t3021 * t2626) * t2625 - t1833 * t2619 + t1701 + t3070 - t2158 * t2626) * t2620 - t1686 * t3798 - (t2174 * t2618 + t3144) * t2619 + t3025 * t3790 - t2624 * t3180 - t2165 * t2626) * t2633 + t1077 * t2634 + t3128;
  C(2,6) = t1095 * t2631 + (((t3006 * t2627 + t4234 * t2626 - 0.1e1 * t3952 + t3145) * t2625 - 0.1e1 * (t3176 + t4227) * t2618) * t2628 + (t2751 * t2625 - 0.1e1 * t2778 * t2618) * t2621 + ((0.13609823097337500000000000000000e-1 * t3793 - 0.1e1 * t2880 * t2618) * t2628 + (t2625 * t2727 + t3836) * t2621) * t2620) * t2632 + t1069 * t2633 + t1062 * t2634 + t1043 * t2635 + t3365;
  C(4,3) = -t1078 * t2633 + t1093 * t2632 + t1102 * t2631 - t3129;
  C(2,1) = t1014 * t2631 + t1012 * t2632 + t1009 * t2633 - 0.1e1 * t1007 * t2634 - 0.1e1 * t1005 * t2635 + (-0.1e1 * t1576 * t3391 + t4324 * t3389 - 0.1e1 * t1736 * t2623 * t4301 - 0.1e1 * (t4338 - 0.1e1 * t3930) * t3391 + (-0.1e1 * t1048 + t1080) * t3805 + (t2143 - 0.1e1 * t4253 - 0.1e1 * t3561) * t2528 * t3536 + (-0.1e1 * t1289 - 0.1e1 * t1400 * t2623 + t4033) * t1389 * t3487 + (t1287 + t1401 * t2630 - 0.1e1 * t4034) * t3397 + (-0.1e1 * t1152 - 0.1e1 * t2556 + (t2621 * t3357 + t4028) * t2630 + (-0.1e1 * t2622 * t3515 - 0.1e1 * t2629 * t3410) * t2623) * t3112 + ((-0.1e1 * t4003 + (-0.1e1 * t4029 - 0.1e1 * t1725 + 0.825e-1) * t2621) * t2623 + (t2629 * t3040 + t3376) * t2630 + t1187) * t3110 - 0.1e1 * (-0.1e1 * (t2871 * t4322 - 0.1e1 * t3866) * t3217 + t3157 * t4349) * t4281 - (-0.1e1 * t1369 * t3488 + (t1572 * t2630 - 0.1e1 * t4019) * t3485) * t1578 + (-0.1e1 * t1354 * t3485 - 0.1e1 * (-0.1e1 * t1520 * t2623 + t4018) * t3488) * t1578 + (-0.50000000000000000000000000000000e0 * t2615 + t4076) * t1051 + (-0.10000000000000000000000000000000e1 * t1767 * t4322 - 0.1e1 * t3116 + t1582) * t1790 * t3486) * t2637;
  C(7,6) = t2846;
  C(4,7) = ((-t2617 * t2820 + t2624 * t2821) * t2619 - (t2626 * t2934 - t3437) * t2617 + (t2626 * t2933 + t3436) * t2624) * t2631 + t1239 * t2632 + t1199 * t2633 + t2946;
  C(1,4) = t1008 * t2636 + t1022 * t2635 + t1033 * t2633 + t1041 * t2632 + t1045 * t2631 + t4057 + ((-t3514 * t2612 * t3784 + ((t1634 * t2625 + t1428) * t2627 + (-t1962 * t3796 + t3137 * t3785 - t1713) * t2620) * t2626 + (t1388 * t3792 + t1577 * t2627 - t1691 * t2620 - t1831) * t2619 + (-t1635 * t2620 - t3072) * t2625 - t1491 * t2620 + t1652 * t2627) * t2622 + (-t2620 * t3522 + t2627 * t3525) * t3788 + ((-t1484 * t2625 + t3511) * t2620 + t3507) * t3824 + t1834 * t3779 + t4109 * t2629) * t2634;
  C(4,5) = t1199 * t2631 + t1185 * t2632 + ((t2625 * t2990 + t2761) * t2626 + (-0.1e1 * t3951 + t3443) * t2619) * t2633 + t2948;
  C(1,2) = t1006 * t2635 + t1008 * t2634 + t1010 * t2633 + t1011 * t2637 + t1013 * t2632 + t1015 * t2631 + (-0.1e1 * t2860 * t3807 * t3817 + t1169 * t2629 * t2614 - 0.1e1 * t3646 * t3935 + t1369 * t1572 * t3485 + (-0.1e1 * t1882 * t2620 * t3795 + 0.1e1 * t3810 * t1599 + t2715 * t3781 - 0.1e1 * t2767 * t3807 + t3075 * t3833 + (-0.1e1 * t1480 * t3657 - 0.1e1 * t2927) * t2622) * t2628 + (t4281 ^ 2 * t3157 + (-0.1e1 * t4183 - 0.1e1 * t2573) * t3389 + (-(-0.1e1 * t4002 - 0.1e1 * t2533 + (-0.316e0 + t3871) * t2629) * t1578 - 0.1e1 * (-0.1e1 * t1732 * t2622 + t2601 + t3035) * t1578) * t3485) * t2623 + 0.70400000000000000000000000000000e-3 * t2622 - 0.1e1 * t2621 * t1527 * t3808 + (-0.15015000000000000000000000000000e-1 + t2798 * t2627 + t2774 * t2620) * t2629 - 0.1e1 * t1354 * (-t4344 - 0.1e1 * t3945) * t3488 + (-0.1e1 * t1351 * t2622 + t2629 * t3375) * t3112 + (-0.1e1 * t1315 * t2622 + t3521 * t3801) * t3110 + t2143 * t2630 * t4272 - 0.1e1 * (-0.3495e-2 * t2623 + t2630 * t3130) * t3130 * t3536 + (-0.1e1 * t3034 - 0.1e1 * t3844) * t3809 + (t2601 + (t4278 + t3131) * t2629) * t2623 * t3397 - (-0.1e1 * t1736 * t3483 + t3217 * t4349) * t2871 + (-0.1e1 * t1582 * t3482 - 0.1e1 * t1576 * t3486) * t1791 + (t1287 * t3487 + t1289 * t3484) * (-t1777 * t2622 + t4250) + (t1152 * t3159 + t1187 * t3219) * (-t1367 * t2622 + t2629 * t3041) + (-0.1e1 * (t3533 - 0.1e1 * t2563) * t2629 - 0.1e1 * t4121) * t2623 * t3391) * t2636;
  C(6,6) = t1698 * t2631;
  C(2,4) = t1072 * t2631 + t1062 * t2632 + t1056 * t2633 + ((-0.1e1 * t1903 * t2625 + t2077) * t3818 + (((-0.1e1 * t1903 - t1932) * t2625 + t2077) * t2626 - 0.1e1 * t2125 * t2625) * t2628 + ((t2619 * t3306 + t2626 * t2813 + 0.1644487577369270e-2) * t2621 + (-t3983 - 0.1e1 * t2170 * t2626 + t2811) * t2628) * t2627 + ((-0.1e1 * t4111 * t3826 - 0.1e1 * t4040 - t4343 + 0.1e1 * t4016 - 0.1e1 * t1834) * t2621 + (0.1e1 * t3971 + 0.50330438027992300000000000000000e0 + (t3199 - 0.1e1 * t2182) * t2618) * t2628) * t2620) * t2634 + t1032 * t2635 + t3367;
  C(6,1) = -t1012 * t2636 - t1029 * t2635 - t1040 * t2634 - t1046 * t2633 + t1063 * t2631 - t4055;
  C(5,3) = t1078 * t2634 + t1106 * t2632 + t1135 * t2631 - t3128;
  C(1,7) = ((-0.1e1 * (-0.1e1 * t2205 * t3786 + t3713) * t2626 * t2617 + (-0.1e1 * t2519 * t2627 * t2617 + (t3713 * t2625 - 0.1e1 * t3878) * t2624) * t2619 + (-0.1e1 * ((-t3341 + t3434) * t2626 + (t2619 * t3016 - t3283 * t3540) * t2625 - t3085) * t2617 + ((-t2627 * t3286 - t3017 - t3342) * t2626 + (t2557 * t3540 - t2619 * t3425) * t2625 + t3086) * t2624) * t2628 + (-0.1e1 * (t3015 * t3793 - 0.1e1 * t3437 * t2627 - t2618 * t4101 + t3437 + (-0.1e1 * t3190 + t3453 + t2949) * t2619) * t2617 + ((t2625 * t2876 + 0.16724826617837780000000000000000e-2) * t2626 + t2618 * t3427 + (0.2444413220184e-2 * t2618 - 0.2580137623800e-3 * t2619) * t2620 + t2619 * t3454 - t3436) * t2624) * t2621) * t2622 - t2707 * t3837 + t2708 * t3799) * t2631 + t1064 * t2632 + t1059 * t2633 + t1045 * t2634 + t1037 * t2635 + t1015 * t2636 + t4053;
  C(6,2) = -t1042 * t2635 - t1061 * t2634 - t1068 * t2633 - t1096 * t2631 - t3365;
  C(4,2) = -t1031 * t2635 - t1057 * t2633 + t1061 * t2632 + t1071 * t2631 - t3367;
  C(6,4) = t1165 * t2633 + t1238 * t2631 - t2947;
  C(7,1) = -t1014 * t2636 - t1036 * t2635 - t1044 * t2634 - t1058 * t2633 - t1063 * t2632 - t4053;
  C(3,6) = t1162 * t2631 + (((-0.1e1 * t4337 + t2451) * t2619 - 0.1e1 * t2003 * t3793) * t2620 + (t2625 * t2790 - t3253) * t2619 + t4314 + ((t3003 + t3242) * t2627 + t4275 * t3791) * t2618) * t2632 + t1107 * t2633 + t1094 * t2634 + t3127;
  C(3,3) = -t1075 * t2634 + t1098 * t2633 + t1099 * t2632 + t1105 * t2631;
end
